simulink model "DualStreamSSR"  (R2023a)
settings: Solver=VariableStepAuto  StartTime=0.0  StopTime=4096  RelTol=1e-3
PreLoadFcn:
  | SSR4_init
InitFcn:
  | SSR4_init
undefined symbols (not defined in the file): DoubleStream, FIR_MultiKernel_cin, FIR_MultiKernel_cincout, FIR_MultiKernel_cout, N, S, SHIFT_ACC, Taps, vsva2197, xcvc1902
libraries: aieBasic x224, aieUtilities x16, dspsrcs4 x1, simulink x1, vmcUtilities x1
(part 2 of 6)

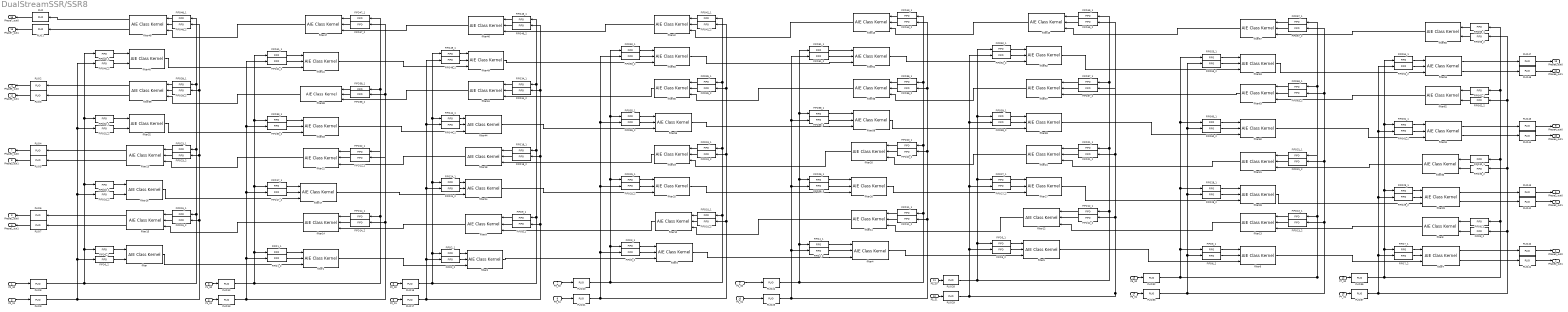
== system DualStreamSSR/SSR8 ==
  P0_S0 : Inport
  P0_S1 : Inport  Port=2
  P1_S0 : Inport  Port=3
  P1_S1 : Inport  Port=4
  P2_S0 : Inport  Port=5
  P2_S1 : Inport  Port=6
  P3_S0 : Inport  Port=7
  P3_S1 : Inport  Port=8
  P4_S0 : Inport  Port=9
  P4_S1 : Inport  Port=10
  P5_S0 : Inport  Port=11
  P5_S1 : Inport  Port=12
  P6_S0 : Inport  Port=13
  P6_S1 : Inport  Port=14
  P7_S0 : Inport  Port=15
  P7_S1 : Inport  Port=16
  FIFO0_1 : aieBasic/FIFO  FifoDepth=512  FIFOType=0  TileType=0  RowLocation=0  ColLocation=0  channel=0  blockJsonConstraints="[{\"type\":\"constraint\",\"constraintType\":\"location_fifo\",\"sid\":\"1153\",\"lhs\":{\"type\":\"location\",\"templParam\":\"fifo\",\"args\":{\"type\":\"fifo\",\"name\":\"DualStreamSSR/SSR8/FIFO0_1\",\"sid\":\"1153\"}},\"rhs\":{\"type\":\"fifogroup\",\"fifotype\":\"dma_fifo\",\"tiletype\":\"aie\",\"column\":{\"type\":\"evaluable\",\"expr\":\"23\",\"value\":23},\"row\":{\"type\":\"evaluable\",\"expr\":\"0\",\"value\":0},\"address\":{\"type\":\"evaluable\",\"expr\":\"0x0000\",\"value\":0},\"identifier\":\"0\",\"size\":{\"type\":\"evaluable\",\"expr\":\"512\",\"value\":512}},\"equality\":true}]"  deprecateConstraints=0
  FIFO0_2 : aieBasic/FIFO  FifoDepth=512  FIFOType=0  TileType=0  RowLocation=0  ColLocation=0  channel=0  blockJsonConstraints="[{\"type\":\"constraint\",\"constraintType\":\"location_fifo\",\"sid\":\"1154\",\"lhs\":{\"type\":\"location\",\"templParam\":\"fifo\",\"args\":{\"type\":\"fifo\",\"name\":\"DualStreamSSR/SSR8/FIFO0_2\",\"sid\":\"1154\"}},\"rhs\":{\"type\":\"fifogroup\",\"fifotype\":\"dma_fifo\",\"tiletype\":\"aie\",\"column\":{\"type\":\"evaluable\",\"expr\":\"23\",\"value\":23},\"row\":{\"type\":\"evaluable\",\"expr\":\"0\",\"value\":0},\"address\":{\"type\":\"evaluable\",\"expr\":\"0x2000\",\"value\":8192},\"identifier\":\"0\",\"size\":{\"type\":\"evaluable\",\"expr\":\"512\",\"value\":512}},\"equality\":true}]"  deprecateConstraints=0
  FIFO10_1 : aieBasic/FIFO  FifoDepth=512  FIFOType=0  TileType=0  RowLocation=0  ColLocation=0  channel=0  blockJsonConstraints="[{\"type\":\"constraint\",\"constraintType\":\"location_fifo\",\"sid\":\"1213\",\"lhs\":{\"type\":\"location\",\"templParam\":\"fifo\",\"args\":{\"type\":\"fifo\",\"name\":\"DualStreamSSR/SSR8/FIFO10_1\",\"sid\":\"1213\"}},\"rhs\":{\"type\":\"fifogroup\",\"fifotype\":\"dma_fifo\",\"tiletype\":\"aie\",\"column\":{\"type\":\"evaluable\",\"expr\":\"26\",\"value\":26},\"row\":{\"type\":\"evaluable\",\"expr\":\"1\",\"value\":1},\"address\":{\"type\":\"evaluable\",\"expr\":\"0x0000\",\"value\":0},\"identifier\":\"0\",\"size\":{\"type\":\"evaluable\",\"expr\":\"512\",\"value\":512}},\"equality\":true}]"  deprecateConstraints=0
  FIFO10_2 : aieBasic/FIFO  FifoDepth=512  FIFOType=0  TileType=0  RowLocation=0  ColLocation=0  channel=0  blockJsonConstraints="[{\"type\":\"constraint\",\"constraintType\":\"location_fifo\",\"sid\":\"1214\",\"lhs\":{\"type\":\"location\",\"templParam\":\"fifo\",\"args\":{\"type\":\"fifo\",\"name\":\"DualStreamSSR/SSR8/FIFO10_2\",\"sid\":\"1214\"}},\"rhs\":{\"type\":\"fifogroup\",\"fifotype\":\"dma_fifo\",\"tiletype\":\"aie\",\"column\":{\"type\":\"evaluable\",\"expr\":\"26\",\"value\":26},\"row\":{\"type\":\"evaluable\",\"expr\":\"1\",\"value\":1},\"address\":{\"type\":\"evaluable\",\"expr\":\"0x2000\",\"value\":8192},\"identifier\":\"0\",\"size\":{\"type\":\"evaluable\",\"expr\":\"512\",\"value\":512}},\"equality\":true}]"  deprecateConstraints=0
  FIFO11_1 : aieBasic/FIFO  FifoDepth=512  FIFOType=0  TileType=0  RowLocation=0  ColLocation=0  channel=0  blockJsonConstraints="[{\"type\":\"constraint\",\"constraintType\":\"location_fifo\",\"sid\":\"1229\",\"lhs\":{\"type\":\"location\",\"templParam\":\"fifo\",\"args\":{\"type\":\"fifo\",\"name\":\"DualStreamSSR/SSR8/FIFO11_1\",\"sid\":\"1229\"}},\"rhs\":{\"type\":\"fifogroup\",\"fifotype\":\"dma_fifo\",\"tiletype\":\"aie\",\"column\":{\"type\":\"evaluable\",\"expr\":\"27\",\"value\":27},\"row\":{\"type\":\"evaluable\",\"expr\":\"1\",\"value\":1},\"address\":{\"type\":\"evaluable\",\"expr\":\"0x0000\",\"value\":0},\"identifier\":\"0\",\"size\":{\"type\":\"evaluable\",\"expr\":\"512\",\"value\":512}},\"equality\":true}]"  deprecateConstraints=0
  FIFO11_2 : aieBasic/FIFO  FifoDepth=512  FIFOType=0  TileType=0  RowLocation=0  ColLocation=0  channel=0  blockJsonConstraints="[{\"type\":\"constraint\",\"constraintType\":\"location_fifo\",\"sid\":\"1230\",\"lhs\":{\"type\":\"location\",\"templParam\":\"fifo\",\"args\":{\"type\":\"fifo\",\"name\":\"DualStreamSSR/SSR8/FIFO11_2\",\"sid\":\"1230\"}},\"rhs\":{\"type\":\"fifogroup\",\"fifotype\":\"dma_fifo\",\"tiletype\":\"aie\",\"column\":{\"type\":\"evaluable\",\"expr\":\"27\",\"value\":27},\"row\":{\"type\":\"evaluable\",\"expr\":\"1\",\"value\":1},\"address\":{\"type\":\"evaluable\",\"expr\":\"0x2000\",\"value\":8192},\"identifier\":\"0\",\"size\":{\"type\":\"evaluable\",\"expr\":\"512\",\"value\":512}},\"equality\":true}]"  deprecateConstraints=0
  FIFO12_1 : aieBasic/FIFO  FifoDepth=512  FIFOType=0  TileType=0  RowLocation=0  ColLocation=0  channel=0  blockJsonConstraints="[{\"type\":\"constraint\",\"constraintType\":\"location_fifo\",\"sid\":\"1245\",\"lhs\":{\"type\":\"location\",\"templParam\":\"fifo\",\"args\":{\"type\":\"fifo\",\"name\":\"DualStreamSSR/SSR8/FIFO12_1\",\"sid\":\"1245\"}},\"rhs\":{\"type\":\"fifogroup\",\"fifotype\":\"dma_fifo\",\"tiletype\":\"aie\",\"column\":{\"type\":\"evaluable\",\"expr\":\"28\",\"value\":28},\"row\":{\"type\":\"evaluable\",\"expr\":\"1\",\"value\":1},\"address\":{\"type\":\"evaluable\",\"expr\":\"0x0000\",\"value\":0},\"identifier\":\"0\",\"size\":{\"type\":\"evaluable\",\"expr\":\"512\",\"value\":512}},\"equality\":true}]"  deprecateConstraints=0
  FIFO12_2 : aieBasic/FIFO  FifoDepth=512  FIFOType=0  TileType=0  RowLocation=0  ColLocation=0  channel=0  blockJsonConstraints="[{\"type\":\"constraint\",\"constraintType\":\"location_fifo\",\"sid\":\"1246\",\"lhs\":{\"type\":\"location\",\"templParam\":\"fifo\",\"args\":{\"type\":\"fifo\",\"name\":\"DualStreamSSR/SSR8/FIFO12_2\",\"sid\":\"1246\"}},\"rhs\":{\"type\":\"fifogroup\",\"fifotype\":\"dma_fifo\",\"tiletype\":\"aie\",\"column\":{\"type\":\"evaluable\",\"expr\":\"28\",\"value\":28},\"row\":{\"type\":\"evaluable\",\"expr\":\"1\",\"value\":1},\"address\":{\"type\":\"evaluable\",\"expr\":\"0x2000\",\"value\":8192},\"identifier\":\"0\",\"size\":{\"type\":\"evaluable\",\"expr\":\"512\",\"value\":512}},\"equality\":true}]"  deprecateConstraints=0
  FIFO13_1 : aieBasic/FIFO  FifoDepth=512  FIFOType=0  TileType=0  RowLocation=0  ColLocation=0  channel=0  blockJsonConstraints="[{\"type\":\"constraint\",\"constraintType\":\"location_fifo\",\"sid\":\"1261\",\"lhs\":{\"type\":\"location\",\"templParam\":\"fifo\",\"args\":{\"type\":\"fifo\",\"name\":\"DualStreamSSR/SSR8/FIFO13_1\",\"sid\":\"1261\"}},\"rhs\":{\"type\":\"fifogroup\",\"fifotype\":\"dma_fifo\",\"tiletype\":\"aie\",\"column\":{\"type\":\"evaluable\",\"expr\":\"29\",\"value\":29},\"row\":{\"type\":\"evaluable\",\"expr\":\"1\",\"value\":1},\"address\":{\"type\":\"evaluable\",\"expr\":\"0x0000\",\"value\":0},\"identifier\":\"0\",\"size\":{\"type\":\"evaluable\",\"expr\":\"512\",\"value\":512}},\"equality\":true}]"  deprecateConstraints=0
  FIFO13_2 : aieBasic/FIFO  FifoDepth=512  FIFOType=0  TileType=0  RowLocation=0  ColLocation=0  channel=0  blockJsonConstraints="[{\"type\":\"constraint\",\"constraintType\":\"location_fifo\",\"sid\":\"1262\",\"lhs\":{\"type\":\"location\",\"templParam\":\"fifo\",\"args\":{\"type\":\"fifo\",\"name\":\"DualStreamSSR/SSR8/FIFO13_2\",\"sid\":\"1262\"}},\"rhs\":{\"type\":\"fifogroup\",\"fifotype\":\"dma_fifo\",\"tiletype\":\"aie\",\"column\":{\"type\":\"evaluable\",\"expr\":\"29\",\"value\":29},\"row\":{\"type\":\"evaluable\",\"expr\":\"1\",\"value\":1},\"address\":{\"type\":\"evaluable\",\"expr\":\"0x2000\",\"value\":8192},\"identifier\":\"0\",\"size\":{\"type\":\"evaluable\",\"expr\":\"512\",\"value\":512}},\"equality\":true}]"  deprecateConstraints=0
  FIFO14_1 : aieBasic/FIFO  FifoDepth=512  FIFOType=0  TileType=0  RowLocation=0  ColLocation=0  channel=0  blockJsonConstraints="[{\"type\":\"constraint\",\"constraintType\":\"location_fifo\",\"sid\":\"1178\",\"lhs\":{\"type\":\"location\",\"templParam\":\"fifo\",\"args\":{\"type\":\"fifo\",\"name\":\"DualStreamSSR/SSR8/FIFO14_1\",\"sid\":\"1178\"}},\"rhs\":{\"type\":\"fifogroup\",\"fifotype\":\"dma_fifo\",\"tiletype\":\"aie\",\"column\":{\"type\":\"evaluable\",\"expr\":\"24\",\"value\":24},\"row\":{\"type\":\"evaluable\",\"expr\":\"1\",\"value\":1},\"address\":{\"type\":\"evaluable\",\"expr\":\"0x0000\",\"value\":0},\"identifier\":\"0\",\"size\":{\"type\":\"evaluable\",\"expr\":\"512\",\"value\":512}},\"equality\":true}]"  deprecateConstraints=0
  FIFO14_2 : aieBasic/FIFO  FifoDepth=512  FIFOType=0  TileType=0  RowLocation=0  ColLocation=0  channel=0  blockJsonConstraints="[{\"type\":\"constraint\",\"constraintType\":\"location_fifo\",\"sid\":\"1179\",\"lhs\":{\"type\":\"location\",\"templParam\":\"fifo\",\"args\":{\"type\":\"fifo\",\"name\":\"DualStreamSSR/SSR8/FIFO14_2\",\"sid\":\"1179\"}},\"rhs\":{\"type\":\"fifogroup\",\"fifotype\":\"dma_fifo\",\"tiletype\":\"aie\",\"column\":{\"type\":\"evaluable\",\"expr\":\"24\",\"value\":24},\"row\":{\"type\":\"evaluable\",\"expr\":\"1\",\"value\":1},\"address\":{\"type\":\"evaluable\",\"expr\":\"0x2000\",\"value\":8192},\"identifier\":\"0\",\"size\":{\"type\":\"evaluable\",\"expr\":\"512\",\"value\":512}},\"equality\":true}]"  deprecateConstraints=0
  FIFO15_1 : aieBasic/FIFO  FifoDepth=512  FIFOType=0  TileType=0  RowLocation=0  ColLocation=0  channel=0  blockJsonConstraints="[{\"type\":\"constraint\",\"constraintType\":\"location_fifo\",\"sid\":\"1162\",\"lhs\":{\"type\":\"location\",\"templParam\":\"fifo\",\"args\":{\"type\":\"fifo\",\"name\":\"DualStreamSSR/SSR8/FIFO15_1\",\"sid\":\"1162\"}},\"rhs\":{\"type\":\"fifogroup\",\"fifotype\":\"dma_fifo\",\"tiletype\":\"aie\",\"column\":{\"type\":\"evaluable\",\"expr\":\"23\",\"value\":23},\"row\":{\"type\":\"evaluable\",\"expr\":\"1\",\"value\":1},\"address\":{\"type\":\"evaluable\",\"expr\":\"0x0000\",\"value\":0},\"identifier\":\"0\",\"size\":{\"type\":\"evaluable\",\"expr\":\"512\",\"value\":512}},\"equality\":true}]"  deprecateConstraints=0
  FIFO15_2 : aieBasic/FIFO  FifoDepth=512  FIFOType=0  TileType=0  RowLocation=0  ColLocation=0  channel=0  blockJsonConstraints="[{\"type\":\"constraint\",\"constraintType\":\"location_fifo\",\"sid\":\"1163\",\"lhs\":{\"type\":\"location\",\"templParam\":\"fifo\",\"args\":{\"type\":\"fifo\",\"name\":\"DualStreamSSR/SSR8/FIFO15_2\",\"sid\":\"1163\"}},\"rhs\":{\"type\":\"fifogroup\",\"fifotype\":\"dma_fifo\",\"tiletype\":\"aie\",\"column\":{\"type\":\"evaluable\",\"expr\":\"23\",\"value\":23},\"row\":{\"type\":\"evaluable\",\"expr\":\"1\",\"value\":1},\"address\":{\"type\":\"evaluable\",\"expr\":\"0x2000\",\"value\":8192},\"identifier\":\"0\",\"size\":{\"type\":\"evaluable\",\"expr\":\"512\",\"value\":512}},\"equality\":true}]"  deprecateConstraints=0
  FIFO16_1 : aieBasic/FIFO  FifoDepth=512  FIFOType=0  TileType=0  RowLocation=0  ColLocation=0  channel=0  blockJsonConstraints="[{\"type\":\"constraint\",\"constraintType\":\"location_fifo\",\"sid\":\"1151\",\"lhs\":{\"type\":\"location\",\"templParam\":\"fifo\",\"args\":{\"type\":\"fifo\",\"name\":\"DualStreamSSR/SSR8/FIFO16_1\",\"sid\":\"1151\"}},\"rhs\":{\"type\":\"fifogroup\",\"fifotype\":\"dma_fifo\",\"tiletype\":\"aie\",\"column\":{\"type\":\"evaluable\",\"expr\":\"23\",\"value\":23},\"row\":{\"type\":\"evaluable\",\"expr\":\"2\",\"value\":2},\"address\":{\"type\":\"evaluable\",\"expr\":\"0x0000\",\"value\":0},\"identifier\":\"0\",\"size\":{\"type\":\"evaluable\",\"expr\":\"512\",\"value\":512}},\"equality\":true}]"  deprecateConstraints=0
  FIFO16_2 : aieBasic/FIFO  FifoDepth=512  FIFOType=0  TileType=0  RowLocation=0  ColLocation=0  channel=0  blockJsonConstraints="[{\"type\":\"constraint\",\"constraintType\":\"location_fifo\",\"sid\":\"1152\",\"lhs\":{\"type\":\"location\",\"templParam\":\"fifo\",\"args\":{\"type\":\"fifo\",\"name\":\"DualStreamSSR/SSR8/FIFO16_2\",\"sid\":\"1152\"}},\"rhs\":{\"type\":\"fifogroup\",\"fifotype\":\"dma_fifo\",\"tiletype\":\"aie\",\"column\":{\"type\":\"evaluable\",\"expr\":\"23\",\"value\":23},\"row\":{\"type\":\"evaluable\",\"expr\":\"2\",\"value\":2},\"address\":{\"type\":\"evaluable\",\"expr\":\"0x2000\",\"value\":8192},\"identifier\":\"0\",\"size\":{\"type\":\"evaluable\",\"expr\":\"512\",\"value\":512}},\"equality\":true}]"  deprecateConstraints=0
  FIFO17_1 : aieBasic/FIFO  FifoDepth=512  FIFOType=0  TileType=0  RowLocation=0  ColLocation=0  channel=0  blockJsonConstraints="[{\"type\":\"constraint\",\"constraintType\":\"location_fifo\",\"sid\":\"1168\",\"lhs\":{\"type\":\"location\",\"templParam\":\"fifo\",\"args\":{\"type\":\"fifo\",\"name\":\"DualStreamSSR/SSR8/FIFO17_1\",\"sid\":\"1168\"}},\"rhs\":{\"type\":\"fifogroup\",\"fifotype\":\"dma_fifo\",\"tiletype\":\"aie\",\"column\":{\"type\":\"evaluable\",\"expr\":\"24\",\"value\":24},\"row\":{\"type\":\"evaluable\",\"expr\":\"2\",\"value\":2},\"address\":{\"type\":\"evaluable\",\"expr\":\"0x0000\",\"value\":0},\"identifier\":\"0\",\"size\":{\"type\":\"evaluable\",\"expr\":\"512\",\"value\":512}},\"equality\":true}]"  deprecateConstraints=0
  FIFO17_2 : aieBasic/FIFO  FifoDepth=512  FIFOType=0  TileType=0  RowLocation=0  ColLocation=0  channel=0  blockJsonConstraints="[{\"type\":\"constraint\",\"constraintType\":\"location_fifo\",\"sid\":\"1169\",\"lhs\":{\"type\":\"location\",\"templParam\":\"fifo\",\"args\":{\"type\":\"fifo\",\"name\":\"DualStreamSSR/SSR8/FIFO17_2\",\"sid\":\"1169\"}},\"rhs\":{\"type\":\"fifogroup\",\"fifotype\":\"dma_fifo\",\"tiletype\":\"aie\",\"column\":{\"type\":\"evaluable\",\"expr\":\"24\",\"value\":24},\"row\":{\"type\":\"evaluable\",\"expr\":\"2\",\"value\":2},\"address\":{\"type\":\"evaluable\",\"expr\":\"0x2000\",\"value\":8192},\"identifier\":\"0\",\"size\":{\"type\":\"evaluable\",\"expr\":\"512\",\"value\":512}},\"equality\":true}]"  deprecateConstraints=0
  FIFO18_1 : aieBasic/FIFO  FifoDepth=512  FIFOType=0  TileType=0  RowLocation=0  ColLocation=0  channel=0  blockJsonConstraints="[{\"type\":\"constraint\",\"constraintType\":\"location_fifo\",\"sid\":\"1193\",\"lhs\":{\"type\":\"location\",\"templParam\":\"fifo\",\"args\":{\"type\":\"fifo\",\"name\":\"DualStreamSSR/SSR8/FIFO18_1\",\"sid\":\"1193\"}},\"rhs\":{\"type\":\"fifogroup\",\"fifotype\":\"dma_fifo\",\"tiletype\":\"aie\",\"column\":{\"type\":\"evaluable\",\"expr\":\"25\",\"value\":25},\"row\":{\"type\":\"evaluable\",\"expr\":\"3\",\"value\":3},\"address\":{\"type\":\"evaluable\",\"expr\":\"0x0000\",\"value\":0},\"identifier\":\"0\",\"size\":{\"type\":\"evaluable\",\"expr\":\"512\",\"value\":512}},\"equality\":true}]"  deprecateConstraints=0
  FIFO18_2 : aieBasic/FIFO  FifoDepth=512  FIFOType=0  TileType=0  RowLocation=0  ColLocation=0  channel=0  blockJsonConstraints="[{\"type\":\"constraint\",\"constraintType\":\"location_fifo\",\"sid\":\"1194\",\"lhs\":{\"type\":\"location\",\"templParam\":\"fifo\",\"args\":{\"type\":\"fifo\",\"name\":\"DualStreamSSR/SSR8/FIFO18_2\",\"sid\":\"1194\"}},\"rhs\":{\"type\":\"fifogroup\",\"fifotype\":\"dma_fifo\",\"tiletype\":\"aie\",\"column\":{\"type\":\"evaluable\",\"expr\":\"25\",\"value\":25},\"row\":{\"type\":\"evaluable\",\"expr\":\"3\",\"value\":3},\"address\":{\"type\":\"evaluable\",\"expr\":\"0x2000\",\"value\":8192},\"identifier\":\"0\",\"size\":{\"type\":\"evaluable\",\"expr\":\"512\",\"value\":512}},\"equality\":true}]"  deprecateConstraints=0
  FIFO19_1 : aieBasic/FIFO  FifoDepth=512  FIFOType=0  TileType=0  RowLocation=0  ColLocation=0  channel=0  blockJsonConstraints="[{\"type\":\"constraint\",\"constraintType\":\"location_fifo\",\"sid\":\"1211\",\"lhs\":{\"type\":\"location\",\"templParam\":\"fifo\",\"args\":{\"type\":\"fifo\",\"name\":\"DualStreamSSR/SSR8/FIFO19_1\",\"sid\":\"1211\"}},\"rhs\":{\"type\":\"fifogroup\",\"fifotype\":\"dma_fifo\",\"tiletype\":\"aie\",\"column\":{\"type\":\"evaluable\",\"expr\":\"26\",\"value\":26},\"row\":{\"type\":\"evaluable\",\"expr\":\"3\",\"value\":3},\"address\":{\"type\":\"evaluable\",\"expr\":\"0x0000\",\"value\":0},\"identifier\":\"0\",\"size\":{\"type\":\"evaluable\",\"expr\":\"512\",\"value\":512}},\"equality\":true}]"  deprecateConstraints=0
  FIFO19_2 : aieBasic/FIFO  FifoDepth=512  FIFOType=0  TileType=0  RowLocation=0  ColLocation=0  channel=0  blockJsonConstraints="[{\"type\":\"constraint\",\"constraintType\":\"location_fifo\",\"sid\":\"1212\",\"lhs\":{\"type\":\"location\",\"templParam\":\"fifo\",\"args\":{\"type\":\"fifo\",\"name\":\"DualStreamSSR/SSR8/FIFO19_2\",\"sid\":\"1212\"}},\"rhs\":{\"type\":\"fifogroup\",\"fifotype\":\"dma_fifo\",\"tiletype\":\"aie\",\"column\":{\"type\":\"evaluable\",\"expr\":\"26\",\"value\":26},\"row\":{\"type\":\"evaluable\",\"expr\":\"3\",\"value\":3},\"address\":{\"type\":\"evaluable\",\"expr\":\"0x2000\",\"value\":8192},\"identifier\":\"0\",\"size\":{\"type\":\"evaluable\",\"expr\":\"512\",\"value\":512}},\"equality\":true}]"  deprecateConstraints=0
  FIFO1_1 : aieBasic/FIFO  FifoDepth=512  FIFOType=0  TileType=0  RowLocation=0  ColLocation=0  channel=0  blockJsonConstraints="[{\"type\":\"constraint\",\"constraintType\":\"location_fifo\",\"sid\":\"1170\",\"lhs\":{\"type\":\"location\",\"templParam\":\"fifo\",\"args\":{\"type\":\"fifo\",\"name\":\"DualStreamSSR/SSR8/FIFO1_1\",\"sid\":\"1170\"}},\"rhs\":{\"type\":\"fifogroup\",\"fifotype\":\"dma_fifo\",\"tiletype\":\"aie\",\"column\":{\"type\":\"evaluable\",\"expr\":\"24\",\"value\":24},\"row\":{\"type\":\"evaluable\",\"expr\":\"0\",\"value\":0},\"address\":{\"type\":\"evaluable\",\"expr\":\"0x0000\",\"value\":0},\"identifier\":\"0\",\"size\":{\"type\":\"evaluable\",\"expr\":\"512\",\"value\":512}},\"equality\":true}]"  deprecateConstraints=0
  FIFO1_2 : aieBasic/FIFO  FifoDepth=512  FIFOType=0  TileType=0  RowLocation=0  ColLocation=0  channel=0  blockJsonConstraints="[{\"type\":\"constraint\",\"constraintType\":\"location_fifo\",\"sid\":\"1171\",\"lhs\":{\"type\":\"location\",\"templParam\":\"fifo\",\"args\":{\"type\":\"fifo\",\"name\":\"DualStreamSSR/SSR8/FIFO1_2\",\"sid\":\"1171\"}},\"rhs\":{\"type\":\"fifogroup\",\"fifotype\":\"dma_fifo\",\"tiletype\":\"aie\",\"column\":{\"type\":\"evaluable\",\"expr\":\"24\",\"value\":24},\"row\":{\"type\":\"evaluable\",\"expr\":\"0\",\"value\":0},\"address\":{\"type\":\"evaluable\",\"expr\":\"0x2000\",\"value\":8192},\"identifier\":\"0\",\"size\":{\"type\":\"evaluable\",\"expr\":\"512\",\"value\":512}},\"equality\":true}]"  deprecateConstraints=0
  FIFO20_1 : aieBasic/FIFO  FifoDepth=512  FIFOType=0  TileType=0  RowLocation=0  ColLocation=0  channel=0  blockJsonConstraints="[{\"type\":\"constraint\",\"constraintType\":\"location_fifo\",\"sid\":\"1227\",\"lhs\":{\"type\":\"location\",\"templParam\":\"fifo\",\"args\":{\"type\":\"fifo\",\"name\":\"DualStreamSSR/SSR8/FIFO20_1\",\"sid\":\"1227\"}},\"rhs\":{\"type\":\"fifogroup\",\"fifotype\":\"dma_fifo\",\"tiletype\":\"aie\",\"column\":{\"type\":\"evaluable\",\"expr\":\"27\",\"value\":27},\"row\":{\"type\":\"evaluable\",\"expr\":\"3\",\"value\":3},\"address\":{\"type\":\"evaluable\",\"expr\":\"0x0000\",\"value\":0},\"identifier\":\"0\",\"size\":{\"type\":\"evaluable\",\"expr\":\"512\",\"value\":512}},\"equality\":true}]"  deprecateConstraints=0
  FIFO20_2 : aieBasic/FIFO  FifoDepth=512  FIFOType=0  TileType=0  RowLocation=0  ColLocation=0  channel=0  blockJsonConstraints="[{\"type\":\"constraint\",\"constraintType\":\"location_fifo\",\"sid\":\"1228\",\"lhs\":{\"type\":\"location\",\"templParam\":\"fifo\",\"args\":{\"type\":\"fifo\",\"name\":\"DualStreamSSR/SSR8/FIFO20_2\",\"sid\":\"1228\"}},\"rhs\":{\"type\":\"fifogroup\",\"fifotype\":\"dma_fifo\",\"tiletype\":\"aie\",\"column\":{\"type\":\"evaluable\",\"expr\":\"27\",\"value\":27},\"row\":{\"type\":\"evaluable\",\"expr\":\"3\",\"value\":3},\"address\":{\"type\":\"evaluable\",\"expr\":\"0x2000\",\"value\":8192},\"identifier\":\"0\",\"size\":{\"type\":\"evaluable\",\"expr\":\"512\",\"value\":512}},\"equality\":true}]"  deprecateConstraints=0
  FIFO21_1 : aieBasic/FIFO  FifoDepth=512  FIFOType=0  TileType=0  RowLocation=0  ColLocation=0  channel=0  blockJsonConstraints="[{\"type\":\"constraint\",\"constraintType\":\"location_fifo\",\"sid\":\"1243\",\"lhs\":{\"type\":\"location\",\"templParam\":\"fifo\",\"args\":{\"type\":\"fifo\",\"name\":\"DualStreamSSR/SSR8/FIFO21_1\",\"sid\":\"1243\"}},\"rhs\":{\"type\":\"fifogroup\",\"fifotype\":\"dma_fifo\",\"tiletype\":\"aie\",\"column\":{\"type\":\"evaluable\",\"expr\":\"28\",\"value\":28},\"row\":{\"type\":\"evaluable\",\"expr\":\"3\",\"value\":3},\"address\":{\"type\":\"evaluable\",\"expr\":\"0x0000\",\"value\":0},\"identifier\":\"0\",\"size\":{\"type\":\"evaluable\",\"expr\":\"512\",\"value\":512}},\"equality\":true}]"  deprecateConstraints=0
  FIFO21_2 : aieBasic/FIFO  FifoDepth=512  FIFOType=0  TileType=0  RowLocation=0  ColLocation=0  channel=0  blockJsonConstraints="[{\"type\":\"constraint\",\"constraintType\":\"location_fifo\",\"sid\":\"1244\",\"lhs\":{\"type\":\"location\",\"templParam\":\"fifo\",\"args\":{\"type\":\"fifo\",\"name\":\"DualStreamSSR/SSR8/FIFO21_2\",\"sid\":\"1244\"}},\"rhs\":{\"type\":\"fifogroup\",\"fifotype\":\"dma_fifo\",\"tiletype\":\"aie\",\"column\":{\"type\":\"evaluable\",\"expr\":\"28\",\"value\":28},\"row\":{\"type\":\"evaluable\",\"expr\":\"3\",\"value\":3},\"address\":{\"type\":\"evaluable\",\"expr\":\"0x2000\",\"value\":8192},\"identifier\":\"0\",\"size\":{\"type\":\"evaluable\",\"expr\":\"512\",\"value\":512}},\"equality\":true}]"  deprecateConstraints=0
  FIFO22_1 : aieBasic/FIFO  FifoDepth=512  FIFOType=0  TileType=0  RowLocation=0  ColLocation=0  channel=0  blockJsonConstraints="[{\"type\":\"constraint\",\"constraintType\":\"location_fifo\",\"sid\":\"1176\",\"lhs\":{\"type\":\"location\",\"templParam\":\"fifo\",\"args\":{\"type\":\"fifo\",\"name\":\"DualStreamSSR/SSR8/FIFO22_1\",\"sid\":\"1176\"}},\"rhs\":{\"type\":\"fifogroup\",\"fifotype\":\"dma_fifo\",\"tiletype\":\"aie\",\"column\":{\"type\":\"evaluable\",\"expr\":\"24\",\"value\":24},\"row\":{\"type\":\"evaluable\",\"expr\":\"3\",\"value\":3},\"address\":{\"type\":\"evaluable\",\"expr\":\"0x0000\",\"value\":0},\"identifier\":\"0\",\"size\":{\"type\":\"evaluable\",\"expr\":\"512\",\"value\":512}},\"equality\":true}]"  deprecateConstraints=0
  FIFO22_2 : aieBasic/FIFO  FifoDepth=512  FIFOType=0  TileType=0  RowLocation=0  ColLocation=0  channel=0  blockJsonConstraints="[{\"type\":\"constraint\",\"constraintType\":\"location_fifo\",\"sid\":\"1177\",\"lhs\":{\"type\":\"location\",\"templParam\":\"fifo\",\"args\":{\"type\":\"fifo\",\"name\":\"DualStreamSSR/SSR8/FIFO22_2\",\"sid\":\"1177\"}},\"rhs\":{\"type\":\"fifogroup\",\"fifotype\":\"dma_fifo\",\"tiletype\":\"aie\",\"column\":{\"type\":\"evaluable\",\"expr\":\"24\",\"value\":24},\"row\":{\"type\":\"evaluable\",\"expr\":\"3\",\"value\":3},\"address\":{\"type\":\"evaluable\",\"expr\":\"0x2000\",\"value\":8192},\"identifier\":\"0\",\"size\":{\"type\":\"evaluable\",\"expr\":\"512\",\"value\":512}},\"equality\":true}]"  deprecateConstraints=0
  FIFO23_1 : aieBasic/FIFO  FifoDepth=512  FIFOType=0  TileType=0  RowLocation=0  ColLocation=0  channel=0  blockJsonConstraints="[{\"type\":\"constraint\",\"constraintType\":\"location_fifo\",\"sid\":\"1160\",\"lhs\":{\"type\":\"location\",\"templParam\":\"fifo\",\"args\":{\"type\":\"fifo\",\"name\":\"DualStreamSSR/SSR8/FIFO23_1\",\"sid\":\"1160\"}},\"rhs\":{\"type\":\"fifogroup\",\"fifotype\":\"dma_fifo\",\"tiletype\":\"aie\",\"column\":{\"type\":\"evaluable\",\"expr\":\"23\",\"value\":23},\"row\":{\"type\":\"evaluable\",\"expr\":\"3\",\"value\":3},\"address\":{\"type\":\"evaluable\",\"expr\":\"0x0000\",\"value\":0},\"identifier\":\"0\",\"size\":{\"type\":\"evaluable\",\"expr\":\"512\",\"value\":512}},\"equality\":true}]"  deprecateConstraints=0
  FIFO23_2 : aieBasic/FIFO  FifoDepth=512  FIFOType=0  TileType=0  RowLocation=0  ColLocation=0  channel=0  blockJsonConstraints="[{\"type\":\"constraint\",\"constraintType\":\"location_fifo\",\"sid\":\"1161\",\"lhs\":{\"type\":\"location\",\"templParam\":\"fifo\",\"args\":{\"type\":\"fifo\",\"name\":\"DualStreamSSR/SSR8/FIFO23_2\",\"sid\":\"1161\"}},\"rhs\":{\"type\":\"fifogroup\",\"fifotype\":\"dma_fifo\",\"tiletype\":\"aie\",\"column\":{\"type\":\"evaluable\",\"expr\":\"23\",\"value\":23},\"row\":{\"type\":\"evaluable\",\"expr\":\"3\",\"value\":3},\"address\":{\"type\":\"evaluable\",\"expr\":\"0x2000\",\"value\":8192},\"identifier\":\"0\",\"size\":{\"type\":\"evaluable\",\"expr\":\"512\",\"value\":512}},\"equality\":true}]"  deprecateConstraints=0
  FIFO24_1 : aieBasic/FIFO  FifoDepth=512  FIFOType=0  TileType=0  RowLocation=0  ColLocation=0  channel=0  blockJsonConstraints="[{\"type\":\"constraint\",\"constraintType\":\"location_fifo\",\"sid\":\"1184\",\"lhs\":{\"type\":\"location\",\"templParam\":\"fifo\",\"args\":{\"type\":\"fifo\",\"name\":\"DualStreamSSR/SSR8/FIFO24_1\",\"sid\":\"1184\"}},\"rhs\":{\"type\":\"fifogroup\",\"fifotype\":\"dma_fifo\",\"tiletype\":\"aie\",\"column\":{\"type\":\"evaluable\",\"expr\":\"25\",\"value\":25},\"row\":{\"type\":\"evaluable\",\"expr\":\"2\",\"value\":2},\"address\":{\"type\":\"evaluable\",\"expr\":\"0x0000\",\"value\":0},\"identifier\":\"0\",\"size\":{\"type\":\"evaluable\",\"expr\":\"512\",\"value\":512}},\"equality\":true}]"  deprecateConstraints=0
  FIFO24_2 : aieBasic/FIFO  FifoDepth=512  FIFOType=0  TileType=0  RowLocation=0  ColLocation=0  channel=0  blockJsonConstraints="[{\"type\":\"constraint\",\"constraintType\":\"location_fifo\",\"sid\":\"1185\",\"lhs\":{\"type\":\"location\",\"templParam\":\"fifo\",\"args\":{\"type\":\"fifo\",\"name\":\"DualStreamSSR/SSR8/FIFO24_2\",\"sid\":\"1185\"}},\"rhs\":{\"type\":\"fifogroup\",\"fifotype\":\"dma_fifo\",\"tiletype\":\"aie\",\"column\":{\"type\":\"evaluable\",\"expr\":\"25\",\"value\":25},\"row\":{\"type\":\"evaluable\",\"expr\":\"2\",\"value\":2},\"address\":{\"type\":\"evaluable\",\"expr\":\"0x2000\",\"value\":8192},\"identifier\":\"0\",\"size\":{\"type\":\"evaluable\",\"expr\":\"512\",\"value\":512}},\"equality\":true}]"  deprecateConstraints=0
  FIFO25_1 : aieBasic/FIFO  FifoDepth=512  FIFOType=0  TileType=0  RowLocation=0  ColLocation=0  channel=0  blockJsonConstraints="[{\"type\":\"constraint\",\"constraintType\":\"location_fifo\",\"sid\":\"1203\",\"lhs\":{\"type\":\"location\",\"templParam\":\"fifo\",\"args\":{\"type\":\"fifo\",\"name\":\"DualStreamSSR/SSR8/FIFO25_1\",\"sid\":\"1203\"}},\"rhs\":{\"type\":\"fifogroup\",\"fifotype\":\"dma_fifo\",\"tiletype\":\"aie\",\"column\":{\"type\":\"evaluable\",\"expr\":\"26\",\"value\":26},\"row\":{\"type\":\"evaluable\",\"expr\":\"2\",\"value\":2},\"address\":{\"type\":\"evaluable\",\"expr\":\"0x0000\",\"value\":0},\"identifier\":\"0\",\"size\":{\"type\":\"evaluable\",\"expr\":\"512\",\"value\":512}},\"equality\":true}]"  deprecateConstraints=0
  FIFO25_2 : aieBasic/FIFO  FifoDepth=512  FIFOType=0  TileType=0  RowLocation=0  ColLocation=0  channel=0  blockJsonConstraints="[{\"type\":\"constraint\",\"constraintType\":\"location_fifo\",\"sid\":\"1204\",\"lhs\":{\"type\":\"location\",\"templParam\":\"fifo\",\"args\":{\"type\":\"fifo\",\"name\":\"DualStreamSSR/SSR8/FIFO25_2\",\"sid\":\"1204\"}},\"rhs\":{\"type\":\"fifogroup\",\"fifotype\":\"dma_fifo\",\"tiletype\":\"aie\",\"column\":{\"type\":\"evaluable\",\"expr\":\"26\",\"value\":26},\"row\":{\"type\":\"evaluable\",\"expr\":\"2\",\"value\":2},\"address\":{\"type\":\"evaluable\",\"expr\":\"0x2000\",\"value\":8192},\"identifier\":\"0\",\"size\":{\"type\":\"evaluable\",\"expr\":\"512\",\"value\":512}},\"equality\":true}]"  deprecateConstraints=0
  FIFO26_1 : aieBasic/FIFO  FifoDepth=512  FIFOType=0  TileType=0  RowLocation=0  ColLocation=0  channel=0  blockJsonConstraints="[{\"type\":\"constraint\",\"constraintType\":\"location_fifo\",\"sid\":\"1219\",\"lhs\":{\"type\":\"location\",\"templParam\":\"fifo\",\"args\":{\"type\":\"fifo\",\"name\":\"DualStreamSSR/SSR8/FIFO26_1\",\"sid\":\"1219\"}},\"rhs\":{\"type\":\"fifogroup\",\"fifotype\":\"dma_fifo\",\"tiletype\":\"aie\",\"column\":{\"type\":\"evaluable\",\"expr\":\"27\",\"value\":27},\"row\":{\"type\":\"evaluable\",\"expr\":\"2\",\"value\":2},\"address\":{\"type\":\"evaluable\",\"expr\":\"0x0000\",\"value\":0},\"identifier\":\"0\",\"size\":{\"type\":\"evaluable\",\"expr\":\"512\",\"value\":512}},\"equality\":true}]"  deprecateConstraints=0
  FIFO26_2 : aieBasic/FIFO  FifoDepth=512  FIFOType=0  TileType=0  RowLocation=0  ColLocation=0  channel=0  blockJsonConstraints="[{\"type\":\"constraint\",\"constraintType\":\"location_fifo\",\"sid\":\"1220\",\"lhs\":{\"type\":\"location\",\"templParam\":\"fifo\",\"args\":{\"type\":\"fifo\",\"name\":\"DualStreamSSR/SSR8/FIFO26_2\",\"sid\":\"1220\"}},\"rhs\":{\"type\":\"fifogroup\",\"fifotype\":\"dma_fifo\",\"tiletype\":\"aie\",\"column\":{\"type\":\"evaluable\",\"expr\":\"27\",\"value\":27},\"row\":{\"type\":\"evaluable\",\"expr\":\"2\",\"value\":2},\"address\":{\"type\":\"evaluable\",\"expr\":\"0x2000\",\"value\":8192},\"identifier\":\"0\",\"size\":{\"type\":\"evaluable\",\"expr\":\"512\",\"value\":512}},\"equality\":true}]"  deprecateConstraints=0
  FIFO27_1 : aieBasic/FIFO  FifoDepth=512  FIFOType=0  TileType=0  RowLocation=0  ColLocation=0  channel=0  blockJsonConstraints="[{\"type\":\"constraint\",\"constraintType\":\"location_fifo\",\"sid\":\"1235\",\"lhs\":{\"type\":\"location\",\"templParam\":\"fifo\",\"args\":{\"type\":\"fifo\",\"name\":\"DualStreamSSR/SSR8/FIFO27_1\",\"sid\":\"1235\"}},\"rhs\":{\"type\":\"fifogroup\",\"fifotype\":\"dma_fifo\",\"tiletype\":\"aie\",\"column\":{\"type\":\"evaluable\",\"expr\":\"28\",\"value\":28},\"row\":{\"type\":\"evaluable\",\"expr\":\"2\",\"value\":2},\"address\":{\"type\":\"evaluable\",\"expr\":\"0x0000\",\"value\":0},\"identifier\":\"0\",\"size\":{\"type\":\"evaluable\",\"expr\":\"512\",\"value\":512}},\"equality\":true}]"  deprecateConstraints=0
  FIFO27_2 : aieBasic/FIFO  FifoDepth=512  FIFOType=0  TileType=0  RowLocation=0  ColLocation=0  channel=0  blockJsonConstraints="[{\"type\":\"constraint\",\"constraintType\":\"location_fifo\",\"sid\":\"1236\",\"lhs\":{\"type\":\"location\",\"templParam\":\"fifo\",\"args\":{\"type\":\"fifo\",\"name\":\"DualStreamSSR/SSR8/FIFO27_2\",\"sid\":\"1236\"}},\"rhs\":{\"type\":\"fifogroup\",\"fifotype\":\"dma_fifo\",\"tiletype\":\"aie\",\"column\":{\"type\":\"evaluable\",\"expr\":\"28\",\"value\":28},\"row\":{\"type\":\"evaluable\",\"expr\":\"2\",\"value\":2},\"address\":{\"type\":\"evaluable\",\"expr\":\"0x2000\",\"value\":8192},\"identifier\":\"0\",\"size\":{\"type\":\"evaluable\",\"expr\":\"512\",\"value\":512}},\"equality\":true}]"  deprecateConstraints=0
  FIFO28_1 : aieBasic/FIFO  FifoDepth=512  FIFOType=0  TileType=0  RowLocation=0  ColLocation=0  channel=0  blockJsonConstraints="[{\"type\":\"constraint\",\"constraintType\":\"location_fifo\",\"sid\":\"1251\",\"lhs\":{\"type\":\"location\",\"templParam\":\"fifo\",\"args\":{\"type\":\"fifo\",\"name\":\"DualStreamSSR/SSR8/FIFO28_1\",\"sid\":\"1251\"}},\"rhs\":{\"type\":\"fifogroup\",\"fifotype\":\"dma_fifo\",\"tiletype\":\"aie\",\"column\":{\"type\":\"evaluable\",\"expr\":\"29\",\"value\":29},\"row\":{\"type\":\"evaluable\",\"expr\":\"2\",\"value\":2},\"address\":{\"type\":\"evaluable\",\"expr\":\"0x0000\",\"value\":0},\"identifier\":\"0\",\"size\":{\"type\":\"evaluable\",\"expr\":\"512\",\"value\":512}},\"equality\":true}]"  deprecateConstraints=0
  FIFO28_2 : aieBasic/FIFO  FifoDepth=512  FIFOType=0  TileType=0  RowLocation=0  ColLocation=0  channel=0  blockJsonConstraints="[{\"type\":\"constraint\",\"constraintType\":\"location_fifo\",\"sid\":\"1252\",\"lhs\":{\"type\":\"location\",\"templParam\":\"fifo\",\"args\":{\"type\":\"fifo\",\"name\":\"DualStreamSSR/SSR8/FIFO28_2\",\"sid\":\"1252\"}},\"rhs\":{\"type\":\"fifogroup\",\"fifotype\":\"dma_fifo\",\"tiletype\":\"aie\",\"column\":{\"type\":\"evaluable\",\"expr\":\"29\",\"value\":29},\"row\":{\"type\":\"evaluable\",\"expr\":\"2\",\"value\":2},\"address\":{\"type\":\"evaluable\",\"expr\":\"0x2000\",\"value\":8192},\"identifier\":\"0\",\"size\":{\"type\":\"evaluable\",\"expr\":\"512\",\"value\":512}},\"equality\":true}]"  deprecateConstraints=0
  FIFO29_1 : aieBasic/FIFO  FifoDepth=512  FIFOType=0  TileType=0  RowLocation=0  ColLocation=0  channel=0  blockJsonConstraints="[{\"type\":\"constraint\",\"constraintType\":\"location_fifo\",\"sid\":\"1267\",\"lhs\":{\"type\":\"location\",\"templParam\":\"fifo\",\"args\":{\"type\":\"fifo\",\"name\":\"DualStreamSSR/SSR8/FIFO29_1\",\"sid\":\"1267\"}},\"rhs\":{\"type\":\"fifogroup\",\"fifotype\":\"dma_fifo\",\"tiletype\":\"aie\",\"column\":{\"type\":\"evaluable\",\"expr\":\"30\",\"value\":30},\"row\":{\"type\":\"evaluable\",\"expr\":\"2\",\"value\":2},\"address\":{\"type\":\"evaluable\",\"expr\":\"0x0000\",\"value\":0},\"identifier\":\"0\",\"size\":{\"type\":\"evaluable\",\"expr\":\"512\",\"value\":512}},\"equality\":true}]"  deprecateConstraints=0
  FIFO29_2 : aieBasic/FIFO  FifoDepth=512  FIFOType=0  TileType=0  RowLocation=0  ColLocation=0  channel=0  blockJsonConstraints="[{\"type\":\"constraint\",\"constraintType\":\"location_fifo\",\"sid\":\"1268\",\"lhs\":{\"type\":\"location\",\"templParam\":\"fifo\",\"args\":{\"type\":\"fifo\",\"name\":\"DualStreamSSR/SSR8/FIFO29_2\",\"sid\":\"1268\"}},\"rhs\":{\"type\":\"fifogroup\",\"fifotype\":\"dma_fifo\",\"tiletype\":\"aie\",\"column\":{\"type\":\"evaluable\",\"expr\":\"30\",\"value\":30},\"row\":{\"type\":\"evaluable\",\"expr\":\"2\",\"value\":2},\"address\":{\"type\":\"evaluable\",\"expr\":\"0x2000\",\"value\":8192},\"identifier\":\"0\",\"size\":{\"type\":\"evaluable\",\"expr\":\"512\",\"value\":512}},\"equality\":true}]"  deprecateConstraints=0
  FIFO2_1 : aieBasic/FIFO  FifoDepth=512  FIFOType=0  TileType=0  RowLocation=0  ColLocation=0  channel=0  blockJsonConstraints="[{\"type\":\"constraint\",\"constraintType\":\"location_fifo\",\"sid\":\"1186\",\"lhs\":{\"type\":\"location\",\"templParam\":\"fifo\",\"args\":{\"type\":\"fifo\",\"name\":\"DualStreamSSR/SSR8/FIFO2_1\",\"sid\":\"1186\"}},\"rhs\":{\"type\":\"fifogroup\",\"fifotype\":\"dma_fifo\",\"tiletype\":\"aie\",\"column\":{\"type\":\"evaluable\",\"expr\":\"25\",\"value\":25},\"row\":{\"type\":\"evaluable\",\"expr\":\"0\",\"value\":0},\"address\":{\"type\":\"evaluable\",\"expr\":\"0x0000\",\"value\":0},\"identifier\":\"0\",\"size\":{\"type\":\"evaluable\",\"expr\":\"512\",\"value\":512}},\"equality\":true}]"  deprecateConstraints=0
  FIFO2_2 : aieBasic/FIFO  FifoDepth=512  FIFOType=0  TileType=0  RowLocation=0  ColLocation=0  channel=0  blockJsonConstraints="[{\"type\":\"constraint\",\"constraintType\":\"location_fifo\",\"sid\":\"1187\",\"lhs\":{\"type\":\"location\",\"templParam\":\"fifo\",\"args\":{\"type\":\"fifo\",\"name\":\"DualStreamSSR/SSR8/FIFO2_2\",\"sid\":\"1187\"}},\"rhs\":{\"type\":\"fifogroup\",\"fifotype\":\"dma_fifo\",\"tiletype\":\"aie\",\"column\":{\"type\":\"evaluable\",\"expr\":\"25\",\"value\":25},\"row\":{\"type\":\"evaluable\",\"expr\":\"0\",\"value\":0},\"address\":{\"type\":\"evaluable\",\"expr\":\"0x2000\",\"value\":8192},\"identifier\":\"0\",\"size\":{\"type\":\"evaluable\",\"expr\":\"512\",\"value\":512}},\"equality\":true}]"  deprecateConstraints=0
  FIFO30_1 : aieBasic/FIFO  FifoDepth=512  FIFOType=0  TileType=0  RowLocation=0  ColLocation=0  channel=0  blockJsonConstraints="[{\"type\":\"constraint\",\"constraintType\":\"location_fifo\",\"sid\":\"1275\",\"lhs\":{\"type\":\"location\",\"templParam\":\"fifo\",\"args\":{\"type\":\"fifo\",\"name\":\"DualStreamSSR/SSR8/FIFO30_1\",\"sid\":\"1275\"}},\"rhs\":{\"type\":\"fifogroup\",\"fifotype\":\"dma_fifo\",\"tiletype\":\"aie\",\"column\":{\"type\":\"evaluable\",\"expr\":\"30\",\"value\":30},\"row\":{\"type\":\"evaluable\",\"expr\":\"3\",\"value\":3},\"address\":{\"type\":\"evaluable\",\"expr\":\"0x0000\",\"value\":0},\"identifier\":\"0\",\"size\":{\"type\":\"evaluable\",\"expr\":\"512\",\"value\":512}},\"equality\":true}]"  deprecateConstraints=0
  FIFO30_2 : aieBasic/FIFO  FifoDepth=512  FIFOType=0  TileType=0  RowLocation=0  ColLocation=0  channel=0  blockJsonConstraints="[{\"type\":\"constraint\",\"constraintType\":\"location_fifo\",\"sid\":\"1276\",\"lhs\":{\"type\":\"location\",\"templParam\":\"fifo\",\"args\":{\"type\":\"fifo\",\"name\":\"DualStreamSSR/SSR8/FIFO30_2\",\"sid\":\"1276\"}},\"rhs\":{\"type\":\"fifogroup\",\"fifotype\":\"dma_fifo\",\"tiletype\":\"aie\",\"column\":{\"type\":\"evaluable\",\"expr\":\"30\",\"value\":30},\"row\":{\"type\":\"evaluable\",\"expr\":\"3\",\"value\":3},\"address\":{\"type\":\"evaluable\",\"expr\":\"0x2000\",\"value\":8192},\"identifier\":\"0\",\"size\":{\"type\":\"evaluable\",\"expr\":\"512\",\"value\":512}},\"equality\":true}]"  deprecateConstraints=0
  FIFO31_1 : aieBasic/FIFO  FifoDepth=512  FIFOType=0  TileType=0  RowLocation=0  ColLocation=0  channel=0  blockJsonConstraints="[{\"type\":\"constraint\",\"constraintType\":\"location_fifo\",\"sid\":\"1259\",\"lhs\":{\"type\":\"location\",\"templParam\":\"fifo\",\"args\":{\"type\":\"fifo\",\"name\":\"DualStreamSSR/SSR8/FIFO31_1\",\"sid\":\"1259\"}},\"rhs\":{\"type\":\"fifogroup\",\"fifotype\":\"dma_fifo\",\"tiletype\":\"aie\",\"column\":{\"type\":\"evaluable\",\"expr\":\"29\",\"value\":29},\"row\":{\"type\":\"evaluable\",\"expr\":\"3\",\"value\":3},\"address\":{\"type\":\"evaluable\",\"expr\":\"0x0000\",\"value\":0},\"identifier\":\"0\",\"size\":{\"type\":\"evaluable\",\"expr\":\"512\",\"value\":512}},\"equality\":true}]"  deprecateConstraints=0
  FIFO31_2 : aieBasic/FIFO  FifoDepth=512  FIFOType=0  TileType=0  RowLocation=0  ColLocation=0  channel=0  blockJsonConstraints="[{\"type\":\"constraint\",\"constraintType\":\"location_fifo\",\"sid\":\"1260\",\"lhs\":{\"type\":\"location\",\"templParam\":\"fifo\",\"args\":{\"type\":\"fifo\",\"name\":\"DualStreamSSR/SSR8/FIFO31_2\",\"sid\":\"1260\"}},\"rhs\":{\"type\":\"fifogroup\",\"fifotype\":\"dma_fifo\",\"tiletype\":\"aie\",\"column\":{\"type\":\"evaluable\",\"expr\":\"29\",\"value\":29},\"row\":{\"type\":\"evaluable\",\"expr\":\"3\",\"value\":3},\"address\":{\"type\":\"evaluable\",\"expr\":\"0x2000\",\"value\":8192},\"identifier\":\"0\",\"size\":{\"type\":\"evaluable\",\"expr\":\"512\",\"value\":512}},\"equality\":true}]"  deprecateConstraints=0
  FIFO32_1 : aieBasic/FIFO  FifoDepth=512  FIFOType=0  TileType=0  RowLocation=0  ColLocation=0  channel=0  blockJsonConstraints="[{\"type\":\"constraint\",\"constraintType\":\"location_fifo\",\"sid\":\"1149\",\"lhs\":{\"type\":\"location\",\"templParam\":\"fifo\",\"args\":{\"type\":\"fifo\",\"name\":\"DualStreamSSR/SSR8/FIFO32_1\",\"sid\":\"1149\"}},\"rhs\":{\"type\":\"fifogroup\",\"fifotype\":\"dma_fifo\",\"tiletype\":\"aie\",\"column\":{\"type\":\"evaluable\",\"expr\":\"23\",\"value\":23},\"row\":{\"type\":\"evaluable\",\"expr\":\"4\",\"value\":4},\"address\":{\"type\":\"evaluable\",\"expr\":\"0x0000\",\"value\":0},\"identifier\":\"0\",\"size\":{\"type\":\"evaluable\",\"expr\":\"512\",\"value\":512}},\"equality\":true}]"  deprecateConstraints=0
  FIFO32_2 : aieBasic/FIFO  FifoDepth=512  FIFOType=0  TileType=0  RowLocation=0  ColLocation=0  channel=0  blockJsonConstraints="[{\"type\":\"constraint\",\"constraintType\":\"location_fifo\",\"sid\":\"1150\",\"lhs\":{\"type\":\"location\",\"templParam\":\"fifo\",\"args\":{\"type\":\"fifo\",\"name\":\"DualStreamSSR/SSR8/FIFO32_2\",\"sid\":\"1150\"}},\"rhs\":{\"type\":\"fifogroup\",\"fifotype\":\"dma_fifo\",\"tiletype\":\"aie\",\"column\":{\"type\":\"evaluable\",\"expr\":\"23\",\"value\":23},\"row\":{\"type\":\"evaluable\",\"expr\":\"4\",\"value\":4},\"address\":{\"type\":\"evaluable\",\"expr\":\"0x2000\",\"value\":8192},\"identifier\":\"0\",\"size\":{\"type\":\"evaluable\",\"expr\":\"512\",\"value\":512}},\"equality\":true}]"  deprecateConstraints=0
  FIFO33_1 : aieBasic/FIFO  FifoDepth=512  FIFOType=0  TileType=0  RowLocation=0  ColLocation=0  channel=0  blockJsonConstraints="[{\"type\":\"constraint\",\"constraintType\":\"location_fifo\",\"sid\":\"1166\",\"lhs\":{\"type\":\"location\",\"templParam\":\"fifo\",\"args\":{\"type\":\"fifo\",\"name\":\"DualStreamSSR/SSR8/FIFO33_1\",\"sid\":\"1166\"}},\"rhs\":{\"type\":\"fifogroup\",\"fifotype\":\"dma_fifo\",\"tiletype\":\"aie\",\"column\":{\"type\":\"evaluable\",\"expr\":\"24\",\"value\":24},\"row\":{\"type\":\"evaluable\",\"expr\":\"4\",\"value\":4},\"address\":{\"type\":\"evaluable\",\"expr\":\"0x0000\",\"value\":0},\"identifier\":\"0\",\"size\":{\"type\":\"evaluable\",\"expr\":\"512\",\"value\":512}},\"equality\":true}]"  deprecateConstraints=0
  FIFO33_2 : aieBasic/FIFO  FifoDepth=512  FIFOType=0  TileType=0  RowLocation=0  ColLocation=0  channel=0  blockJsonConstraints="[{\"type\":\"constraint\",\"constraintType\":\"location_fifo\",\"sid\":\"1167\",\"lhs\":{\"type\":\"location\",\"templParam\":\"fifo\",\"args\":{\"type\":\"fifo\",\"name\":\"DualStreamSSR/SSR8/FIFO33_2\",\"sid\":\"1167\"}},\"rhs\":{\"type\":\"fifogroup\",\"fifotype\":\"dma_fifo\",\"tiletype\":\"aie\",\"column\":{\"type\":\"evaluable\",\"expr\":\"24\",\"value\":24},\"row\":{\"type\":\"evaluable\",\"expr\":\"4\",\"value\":4},\"address\":{\"type\":\"evaluable\",\"expr\":\"0x2000\",\"value\":8192},\"identifier\":\"0\",\"size\":{\"type\":\"evaluable\",\"expr\":\"512\",\"value\":512}},\"equality\":true}]"  deprecateConstraints=0
  FIFO34_1 : aieBasic/FIFO  FifoDepth=512  FIFOType=0  TileType=0  RowLocation=0  ColLocation=0  channel=0  blockJsonConstraints="[{\"type\":\"constraint\",\"constraintType\":\"location_fifo\",\"sid\":\"1191\",\"lhs\":{\"type\":\"location\",\"templParam\":\"fifo\",\"args\":{\"type\":\"fifo\",\"name\":\"DualStreamSSR/SSR8/FIFO34_1\",\"sid\":\"1191\"}},\"rhs\":{\"type\":\"fifogroup\",\"fifotype\":\"dma_fifo\",\"tiletype\":\"aie\",\"column\":{\"type\":\"evaluable\",\"expr\":\"25\",\"value\":25},\"row\":{\"type\":\"evaluable\",\"expr\":\"5\",\"value\":5},\"address\":{\"type\":\"evaluable\",\"expr\":\"0x0000\",\"value\":0},\"identifier\":\"0\",\"size\":{\"type\":\"evaluable\",\"expr\":\"512\",\"value\":512}},\"equality\":true}]"  deprecateConstraints=0
  FIFO34_2 : aieBasic/FIFO  FifoDepth=512  FIFOType=0  TileType=0  RowLocation=0  ColLocation=0  channel=0  blockJsonConstraints="[{\"type\":\"constraint\",\"constraintType\":\"location_fifo\",\"sid\":\"1192\",\"lhs\":{\"type\":\"location\",\"templParam\":\"fifo\",\"args\":{\"type\":\"fifo\",\"name\":\"DualStreamSSR/SSR8/FIFO34_2\",\"sid\":\"1192\"}},\"rhs\":{\"type\":\"fifogroup\",\"fifotype\":\"dma_fifo\",\"tiletype\":\"aie\",\"column\":{\"type\":\"evaluable\",\"expr\":\"25\",\"value\":25},\"row\":{\"type\":\"evaluable\",\"expr\":\"5\",\"value\":5},\"address\":{\"type\":\"evaluable\",\"expr\":\"0x2000\",\"value\":8192},\"identifier\":\"0\",\"size\":{\"type\":\"evaluable\",\"expr\":\"512\",\"value\":512}},\"equality\":true}]"  deprecateConstraints=0
  FIFO35_1 : aieBasic/FIFO  FifoDepth=512  FIFOType=0  TileType=0  RowLocation=0  ColLocation=0  channel=0  blockJsonConstraints="[{\"type\":\"constraint\",\"constraintType\":\"location_fifo\",\"sid\":\"1209\",\"lhs\":{\"type\":\"location\",\"templParam\":\"fifo\",\"args\":{\"type\":\"fifo\",\"name\":\"DualStreamSSR/SSR8/FIFO35_1\",\"sid\":\"1209\"}},\"rhs\":{\"type\":\"fifogroup\",\"fifotype\":\"dma_fifo\",\"tiletype\":\"aie\",\"column\":{\"type\":\"evaluable\",\"expr\":\"26\",\"value\":26},\"row\":{\"type\":\"evaluable\",\"expr\":\"5\",\"value\":5},\"address\":{\"type\":\"evaluable\",\"expr\":\"0x0000\",\"value\":0},\"identifier\":\"0\",\"size\":{\"type\":\"evaluable\",\"expr\":\"512\",\"value\":512}},\"equality\":true}]"  deprecateConstraints=0
  FIFO35_2 : aieBasic/FIFO  FifoDepth=512  FIFOType=0  TileType=0  RowLocation=0  ColLocation=0  channel=0  blockJsonConstraints="[{\"type\":\"constraint\",\"constraintType\":\"location_fifo\",\"sid\":\"1210\",\"lhs\":{\"type\":\"location\",\"templParam\":\"fifo\",\"args\":{\"type\":\"fifo\",\"name\":\"DualStreamSSR/SSR8/FIFO35_2\",\"sid\":\"1210\"}},\"rhs\":{\"type\":\"fifogroup\",\"fifotype\":\"dma_fifo\",\"tiletype\":\"aie\",\"column\":{\"type\":\"evaluable\",\"expr\":\"26\",\"value\":26},\"row\":{\"type\":\"evaluable\",\"expr\":\"5\",\"value\":5},\"address\":{\"type\":\"evaluable\",\"expr\":\"0x2000\",\"value\":8192},\"identifier\":\"0\",\"size\":{\"type\":\"evaluable\",\"expr\":\"512\",\"value\":512}},\"equality\":true}]"  deprecateConstraints=0
  FIFO36_1 : aieBasic/FIFO  FifoDepth=512  FIFOType=0  TileType=0  RowLocation=0  ColLocation=0  channel=0  blockJsonConstraints="[{\"type\":\"constraint\",\"constraintType\":\"location_fifo\",\"sid\":\"1225\",\"lhs\":{\"type\":\"location\",\"templParam\":\"fifo\",\"args\":{\"type\":\"fifo\",\"name\":\"DualStreamSSR/SSR8/FIFO36_1\",\"sid\":\"1225\"}},\"rhs\":{\"type\":\"fifogroup\",\"fifotype\":\"dma_fifo\",\"tiletype\":\"aie\",\"column\":{\"type\":\"evaluable\",\"expr\":\"27\",\"value\":27},\"row\":{\"type\":\"evaluable\",\"expr\":\"5\",\"value\":5},\"address\":{\"type\":\"evaluable\",\"expr\":\"0x0000\",\"value\":0},\"identifier\":\"0\",\"size\":{\"type\":\"evaluable\",\"expr\":\"512\",\"value\":512}},\"equality\":true}]"  deprecateConstraints=0
  FIFO36_2 : aieBasic/FIFO  FifoDepth=512  FIFOType=0  TileType=0  RowLocation=0  ColLocation=0  channel=0  blockJsonConstraints="[{\"type\":\"constraint\",\"constraintType\":\"location_fifo\",\"sid\":\"1226\",\"lhs\":{\"type\":\"location\",\"templParam\":\"fifo\",\"args\":{\"type\":\"fifo\",\"name\":\"DualStreamSSR/SSR8/FIFO36_2\",\"sid\":\"1226\"}},\"rhs\":{\"type\":\"fifogroup\",\"fifotype\":\"dma_fifo\",\"tiletype\":\"aie\",\"column\":{\"type\":\"evaluable\",\"expr\":\"27\",\"value\":27},\"row\":{\"type\":\"evaluable\",\"expr\":\"5\",\"value\":5},\"address\":{\"type\":\"evaluable\",\"expr\":\"0x2000\",\"value\":8192},\"identifier\":\"0\",\"size\":{\"type\":\"evaluable\",\"expr\":\"512\",\"value\":512}},\"equality\":true}]"  deprecateConstraints=0
  FIFO37_1 : aieBasic/FIFO  FifoDepth=512  FIFOType=0  TileType=0  RowLocation=0  ColLocation=0  channel=0  blockJsonConstraints="[{\"type\":\"constraint\",\"constraintType\":\"location_fifo\",\"sid\":\"1241\",\"lhs\":{\"type\":\"location\",\"templParam\":\"fifo\",\"args\":{\"type\":\"fifo\",\"name\":\"DualStreamSSR/SSR8/FIFO37_1\",\"sid\":\"1241\"}},\"rhs\":{\"type\":\"fifogroup\",\"fifotype\":\"dma_fifo\",\"tiletype\":\"aie\",\"column\":{\"type\":\"evaluable\",\"expr\":\"28\",\"value\":28},\"row\":{\"type\":\"evaluable\",\"expr\":\"5\",\"value\":5},\"address\":{\"type\":\"evaluable\",\"expr\":\"0x0000\",\"value\":0},\"identifier\":\"0\",\"size\":{\"type\":\"evaluable\",\"expr\":\"512\",\"value\":512}},\"equality\":true}]"  deprecateConstraints=0
  FIFO37_2 : aieBasic/FIFO  FifoDepth=512  FIFOType=0  TileType=0  RowLocation=0  ColLocation=0  channel=0  blockJsonConstraints="[{\"type\":\"constraint\",\"constraintType\":\"location_fifo\",\"sid\":\"1242\",\"lhs\":{\"type\":\"location\",\"templParam\":\"fifo\",\"args\":{\"type\":\"fifo\",\"name\":\"DualStreamSSR/SSR8/FIFO37_2\",\"sid\":\"1242\"}},\"rhs\":{\"type\":\"fifogroup\",\"fifotype\":\"dma_fifo\",\"tiletype\":\"aie\",\"column\":{\"type\":\"evaluable\",\"expr\":\"28\",\"value\":28},\"row\":{\"type\":\"evaluable\",\"expr\":\"5\",\"value\":5},\"address\":{\"type\":\"evaluable\",\"expr\":\"0x2000\",\"value\":8192},\"identifier\":\"0\",\"size\":{\"type\":\"evaluable\",\"expr\":\"512\",\"value\":512}},\"equality\":true}]"  deprecateConstraints=0
  FIFO38_1 : aieBasic/FIFO  FifoDepth=512  FIFOType=0  TileType=0  RowLocation=0  ColLocation=0  channel=0  blockJsonConstraints="[{\"type\":\"constraint\",\"constraintType\":\"location_fifo\",\"sid\":\"1174\",\"lhs\":{\"type\":\"location\",\"templParam\":\"fifo\",\"args\":{\"type\":\"fifo\",\"name\":\"DualStreamSSR/SSR8/FIFO38_1\",\"sid\":\"1174\"}},\"rhs\":{\"type\":\"fifogroup\",\"fifotype\":\"dma_fifo\",\"tiletype\":\"aie\",\"column\":{\"type\":\"evaluable\",\"expr\":\"24\",\"value\":24},\"row\":{\"type\":\"evaluable\",\"expr\":\"5\",\"value\":5},\"address\":{\"type\":\"evaluable\",\"expr\":\"0x0000\",\"value\":0},\"identifier\":\"0\",\"size\":{\"type\":\"evaluable\",\"expr\":\"512\",\"value\":512}},\"equality\":true}]"  deprecateConstraints=0
  FIFO38_2 : aieBasic/FIFO  FifoDepth=512  FIFOType=0  TileType=0  RowLocation=0  ColLocation=0  channel=0  blockJsonConstraints="[{\"type\":\"constraint\",\"constraintType\":\"location_fifo\",\"sid\":\"1175\",\"lhs\":{\"type\":\"location\",\"templParam\":\"fifo\",\"args\":{\"type\":\"fifo\",\"name\":\"DualStreamSSR/SSR8/FIFO38_2\",\"sid\":\"1175\"}},\"rhs\":{\"type\":\"fifogroup\",\"fifotype\":\"dma_fifo\",\"tiletype\":\"aie\",\"column\":{\"type\":\"evaluable\",\"expr\":\"24\",\"value\":24},\"row\":{\"type\":\"evaluable\",\"expr\":\"5\",\"value\":5},\"address\":{\"type\":\"evaluable\",\"expr\":\"0x2000\",\"value\":8192},\"identifier\":\"0\",\"size\":{\"type\":\"evaluable\",\"expr\":\"512\",\"value\":512}},\"equality\":true}]"  deprecateConstraints=0
  FIFO39_1 : aieBasic/FIFO  FifoDepth=512  FIFOType=0  TileType=0  RowLocation=0  ColLocation=0  channel=0  blockJsonConstraints="[{\"type\":\"constraint\",\"constraintType\":\"location_fifo\",\"sid\":\"1158\",\"lhs\":{\"type\":\"location\",\"templParam\":\"fifo\",\"args\":{\"type\":\"fifo\",\"name\":\"DualStreamSSR/SSR8/FIFO39_1\",\"sid\":\"1158\"}},\"rhs\":{\"type\":\"fifogroup\",\"fifotype\":\"dma_fifo\",\"tiletype\":\"aie\",\"column\":{\"type\":\"evaluable\",\"expr\":\"23\",\"value\":23},\"row\":{\"type\":\"evaluable\",\"expr\":\"5\",\"value\":5},\"address\":{\"type\":\"evaluable\",\"expr\":\"0x0000\",\"value\":0},\"identifier\":\"0\",\"size\":{\"type\":\"evaluable\",\"expr\":\"512\",\"value\":512}},\"equality\":true}]"  deprecateConstraints=0
  FIFO39_2 : aieBasic/FIFO  FifoDepth=512  FIFOType=0  TileType=0  RowLocation=0  ColLocation=0  channel=0  blockJsonConstraints="[{\"type\":\"constraint\",\"constraintType\":\"location_fifo\",\"sid\":\"1159\",\"lhs\":{\"type\":\"location\",\"templParam\":\"fifo\",\"args\":{\"type\":\"fifo\",\"name\":\"DualStreamSSR/SSR8/FIFO39_2\",\"sid\":\"1159\"}},\"rhs\":{\"type\":\"fifogroup\",\"fifotype\":\"dma_fifo\",\"tiletype\":\"aie\",\"column\":{\"type\":\"evaluable\",\"expr\":\"23\",\"value\":23},\"row\":{\"type\":\"evaluable\",\"expr\":\"5\",\"value\":5},\"address\":{\"type\":\"evaluable\",\"expr\":\"0x2000\",\"value\":8192},\"identifier\":\"0\",\"size\":{\"type\":\"evaluable\",\"expr\":\"512\",\"value\":512}},\"equality\":true}]"  deprecateConstraints=0
  FIFO3_1 : aieBasic/FIFO  FifoDepth=512  FIFOType=0  TileType=0  RowLocation=0  ColLocation=0  channel=0  blockJsonConstraints="[{\"type\":\"constraint\",\"constraintType\":\"location_fifo\",\"sid\":\"1205\",\"lhs\":{\"type\":\"location\",\"templParam\":\"fifo\",\"args\":{\"type\":\"fifo\",\"name\":\"DualStreamSSR/SSR8/FIFO3_1\",\"sid\":\"1205\"}},\"rhs\":{\"type\":\"fifogroup\",\"fifotype\":\"dma_fifo\",\"tiletype\":\"aie\",\"column\":{\"type\":\"evaluable\",\"expr\":\"26\",\"value\":26},\"row\":{\"type\":\"evaluable\",\"expr\":\"0\",\"value\":0},\"address\":{\"type\":\"evaluable\",\"expr\":\"0x0000\",\"value\":0},\"identifier\":\"0\",\"size\":{\"type\":\"evaluable\",\"expr\":\"512\",\"value\":512}},\"equality\":true}]"  deprecateConstraints=0
  FIFO3_2 : aieBasic/FIFO  FifoDepth=512  FIFOType=0  TileType=0  RowLocation=0  ColLocation=0  channel=0  blockJsonConstraints="[{\"type\":\"constraint\",\"constraintType\":\"location_fifo\",\"sid\":\"1206\",\"lhs\":{\"type\":\"location\",\"templParam\":\"fifo\",\"args\":{\"type\":\"fifo\",\"name\":\"DualStreamSSR/SSR8/FIFO3_2\",\"sid\":\"1206\"}},\"rhs\":{\"type\":\"fifogroup\",\"fifotype\":\"dma_fifo\",\"tiletype\":\"aie\",\"column\":{\"type\":\"evaluable\",\"expr\":\"26\",\"value\":26},\"row\":{\"type\":\"evaluable\",\"expr\":\"0\",\"value\":0},\"address\":{\"type\":\"evaluable\",\"expr\":\"0x2000\",\"value\":8192},\"identifier\":\"0\",\"size\":{\"type\":\"evaluable\",\"expr\":\"512\",\"value\":512}},\"equality\":true}]"  deprecateConstraints=0
  FIFO40_1 : aieBasic/FIFO  FifoDepth=512  FIFOType=0  TileType=0  RowLocation=0  ColLocation=0  channel=0  blockJsonConstraints="[{\"type\":\"constraint\",\"constraintType\":\"location_fifo\",\"sid\":\"1147\",\"lhs\":{\"type\":\"location\",\"templParam\":\"fifo\",\"args\":{\"type\":\"fifo\",\"name\":\"DualStreamSSR/SSR8/FIFO40_1\",\"sid\":\"1147\"}},\"rhs\":{\"type\":\"fifogroup\",\"fifotype\":\"dma_fifo\",\"tiletype\":\"aie\",\"column\":{\"type\":\"evaluable\",\"expr\":\"23\",\"value\":23},\"row\":{\"type\":\"evaluable\",\"expr\":\"6\",\"value\":6},\"address\":{\"type\":\"evaluable\",\"expr\":\"0x0000\",\"value\":0},\"identifier\":\"0\",\"size\":{\"type\":\"evaluable\",\"expr\":\"512\",\"value\":512}},\"equality\":true}]"  deprecateConstraints=0
  FIFO40_2 : aieBasic/FIFO  FifoDepth=512  FIFOType=0  TileType=0  RowLocation=0  ColLocation=0  channel=0  blockJsonConstraints="[{\"type\":\"constraint\",\"constraintType\":\"location_fifo\",\"sid\":\"1148\",\"lhs\":{\"type\":\"location\",\"templParam\":\"fifo\",\"args\":{\"type\":\"fifo\",\"name\":\"DualStreamSSR/SSR8/FIFO40_2\",\"sid\":\"1148\"}},\"rhs\":{\"type\":\"fifogroup\",\"fifotype\":\"dma_fifo\",\"tiletype\":\"aie\",\"column\":{\"type\":\"evaluable\",\"expr\":\"23\",\"value\":23},\"row\":{\"type\":\"evaluable\",\"expr\":\"6\",\"value\":6},\"address\":{\"type\":\"evaluable\",\"expr\":\"0x2000\",\"value\":8192},\"identifier\":\"0\",\"size\":{\"type\":\"evaluable\",\"expr\":\"512\",\"value\":512}},\"equality\":true}]"  deprecateConstraints=0
  FIFO41_1 : aieBasic/FIFO  FifoDepth=512  FIFOType=0  TileType=0  RowLocation=0  ColLocation=0  channel=0  blockJsonConstraints="[{\"type\":\"constraint\",\"constraintType\":\"location_fifo\",\"sid\":\"1164\",\"lhs\":{\"type\":\"location\",\"templParam\":\"fifo\",\"args\":{\"type\":\"fifo\",\"name\":\"DualStreamSSR/SSR8/FIFO41_1\",\"sid\":\"1164\"}},\"rhs\":{\"type\":\"fifogroup\",\"fifotype\":\"dma_fifo\",\"tiletype\":\"aie\",\"column\":{\"type\":\"evaluable\",\"expr\":\"24\",\"value\":24},\"row\":{\"type\":\"evaluable\",\"expr\":\"6\",\"value\":6},\"address\":{\"type\":\"evaluable\",\"expr\":\"0x0000\",\"value\":0},\"identifier\":\"0\",\"size\":{\"type\":\"evaluable\",\"expr\":\"512\",\"value\":512}},\"equality\":true}]"  deprecateConstraints=0
  FIFO41_2 : aieBasic/FIFO  FifoDepth=512  FIFOType=0  TileType=0  RowLocation=0  ColLocation=0  channel=0  blockJsonConstraints="[{\"type\":\"constraint\",\"constraintType\":\"location_fifo\",\"sid\":\"1165\",\"lhs\":{\"type\":\"location\",\"templParam\":\"fifo\",\"args\":{\"type\":\"fifo\",\"name\":\"DualStreamSSR/SSR8/FIFO41_2\",\"sid\":\"1165\"}},\"rhs\":{\"type\":\"fifogroup\",\"fifotype\":\"dma_fifo\",\"tiletype\":\"aie\",\"column\":{\"type\":\"evaluable\",\"expr\":\"24\",\"value\":24},\"row\":{\"type\":\"evaluable\",\"expr\":\"6\",\"value\":6},\"address\":{\"type\":\"evaluable\",\"expr\":\"0x2000\",\"value\":8192},\"identifier\":\"0\",\"size\":{\"type\":\"evaluable\",\"expr\":\"512\",\"value\":512}},\"equality\":true}]"  deprecateConstraints=0
  FIFO42_1 : aieBasic/FIFO  FifoDepth=512  FIFOType=0  TileType=0  RowLocation=0  ColLocation=0  channel=0  blockJsonConstraints="[{\"type\":\"constraint\",\"constraintType\":\"location_fifo\",\"sid\":\"1207\",\"lhs\":{\"type\":\"location\",\"templParam\":\"fifo\",\"args\":{\"type\":\"fifo\",\"name\":\"DualStreamSSR/SSR8/FIFO42_1\",\"sid\":\"1207\"}},\"rhs\":{\"type\":\"fifogroup\",\"fifotype\":\"dma_fifo\",\"tiletype\":\"aie\",\"column\":{\"type\":\"evaluable\",\"expr\":\"26\",\"value\":26},\"row\":{\"type\":\"evaluable\",\"expr\":\"7\",\"value\":7},\"address\":{\"type\":\"evaluable\",\"expr\":\"0x0000\",\"value\":0},\"identifier\":\"0\",\"size\":{\"type\":\"evaluable\",\"expr\":\"512\",\"value\":512}},\"equality\":true}]"  deprecateConstraints=0
  FIFO42_2 : aieBasic/FIFO  FifoDepth=512  FIFOType=0  TileType=0  RowLocation=0  ColLocation=0  channel=0  blockJsonConstraints="[{\"type\":\"constraint\",\"constraintType\":\"location_fifo\",\"sid\":\"1208\",\"lhs\":{\"type\":\"location\",\"templParam\":\"fifo\",\"args\":{\"type\":\"fifo\",\"name\":\"DualStreamSSR/SSR8/FIFO42_2\",\"sid\":\"1208\"}},\"rhs\":{\"type\":\"fifogroup\",\"fifotype\":\"dma_fifo\",\"tiletype\":\"aie\",\"column\":{\"type\":\"evaluable\",\"expr\":\"26\",\"value\":26},\"row\":{\"type\":\"evaluable\",\"expr\":\"7\",\"value\":7},\"address\":{\"type\":\"evaluable\",\"expr\":\"0x2000\",\"value\":8192},\"identifier\":\"0\",\"size\":{\"type\":\"evaluable\",\"expr\":\"512\",\"value\":512}},\"equality\":true}]"  deprecateConstraints=0
  FIFO43_1 : aieBasic/FIFO  FifoDepth=512  FIFOType=0  TileType=0  RowLocation=0  ColLocation=0  channel=0  blockJsonConstraints="[{\"type\":\"constraint\",\"constraintType\":\"location_fifo\",\"sid\":\"1223\",\"lhs\":{\"type\":\"location\",\"templParam\":\"fifo\",\"args\":{\"type\":\"fifo\",\"name\":\"DualStreamSSR/SSR8/FIFO43_1\",\"sid\":\"1223\"}},\"rhs\":{\"type\":\"fifogroup\",\"fifotype\":\"dma_fifo\",\"tiletype\":\"aie\",\"column\":{\"type\":\"evaluable\",\"expr\":\"27\",\"value\":27},\"row\":{\"type\":\"evaluable\",\"expr\":\"7\",\"value\":7},\"address\":{\"type\":\"evaluable\",\"expr\":\"0x0000\",\"value\":0},\"identifier\":\"0\",\"size\":{\"type\":\"evaluable\",\"expr\":\"512\",\"value\":512}},\"equality\":true}]"  deprecateConstraints=0
  FIFO43_2 : aieBasic/FIFO  FifoDepth=512  FIFOType=0  TileType=0  RowLocation=0  ColLocation=0  channel=0  blockJsonConstraints="[{\"type\":\"constraint\",\"constraintType\":\"location_fifo\",\"sid\":\"1224\",\"lhs\":{\"type\":\"location\",\"templParam\":\"fifo\",\"args\":{\"type\":\"fifo\",\"name\":\"DualStreamSSR/SSR8/FIFO43_2\",\"sid\":\"1224\"}},\"rhs\":{\"type\":\"fifogroup\",\"fifotype\":\"dma_fifo\",\"tiletype\":\"aie\",\"column\":{\"type\":\"evaluable\",\"expr\":\"27\",\"value\":27},\"row\":{\"type\":\"evaluable\",\"expr\":\"7\",\"value\":7},\"address\":{\"type\":\"evaluable\",\"expr\":\"0x2000\",\"value\":8192},\"identifier\":\"0\",\"size\":{\"type\":\"evaluable\",\"expr\":\"512\",\"value\":512}},\"equality\":true}]"  deprecateConstraints=0
  FIFO44_1 : aieBasic/FIFO  FifoDepth=512  FIFOType=0  TileType=0  RowLocation=0  ColLocation=0  channel=0  blockJsonConstraints="[{\"type\":\"constraint\",\"constraintType\":\"location_fifo\",\"sid\":\"1182\",\"lhs\":{\"type\":\"location\",\"templParam\":\"fifo\",\"args\":{\"type\":\"fifo\",\"name\":\"DualStreamSSR/SSR8/FIFO44_1\",\"sid\":\"1182\"}},\"rhs\":{\"type\":\"fifogroup\",\"fifotype\":\"dma_fifo\",\"tiletype\":\"aie\",\"column\":{\"type\":\"evaluable\",\"expr\":\"25\",\"value\":25},\"row\":{\"type\":\"evaluable\",\"expr\":\"4\",\"value\":4},\"address\":{\"type\":\"evaluable\",\"expr\":\"0x0000\",\"value\":0},\"identifier\":\"0\",\"size\":{\"type\":\"evaluable\",\"expr\":\"512\",\"value\":512}},\"equality\":true}]"  deprecateConstraints=0
  FIFO44_2 : aieBasic/FIFO  FifoDepth=512  FIFOType=0  TileType=0  RowLocation=0  ColLocation=0  channel=0  blockJsonConstraints="[{\"type\":\"constraint\",\"constraintType\":\"location_fifo\",\"sid\":\"1183\",\"lhs\":{\"type\":\"location\",\"templParam\":\"fifo\",\"args\":{\"type\":\"fifo\",\"name\":\"DualStreamSSR/SSR8/FIFO44_2\",\"sid\":\"1183\"}},\"rhs\":{\"type\":\"fifogroup\",\"fifotype\":\"dma_fifo\",\"tiletype\":\"aie\",\"column\":{\"type\":\"evaluable\",\"expr\":\"25\",\"value\":25},\"row\":{\"type\":\"evaluable\",\"expr\":\"4\",\"value\":4},\"address\":{\"type\":\"evaluable\",\"expr\":\"0x2000\",\"value\":8192},\"identifier\":\"0\",\"size\":{\"type\":\"evaluable\",\"expr\":\"512\",\"value\":512}},\"equality\":true}]"  deprecateConstraints=0
  FIFO45_1 : aieBasic/FIFO  FifoDepth=512  FIFOType=0  TileType=0  RowLocation=0  ColLocation=0  channel=0  blockJsonConstraints="[{\"type\":\"constraint\",\"constraintType\":\"location_fifo\",\"sid\":\"1239\",\"lhs\":{\"type\":\"location\",\"templParam\":\"fifo\",\"args\":{\"type\":\"fifo\",\"name\":\"DualStreamSSR/SSR8/FIFO45_1\",\"sid\":\"1239\"}},\"rhs\":{\"type\":\"fifogroup\",\"fifotype\":\"dma_fifo\",\"tiletype\":\"aie\",\"column\":{\"type\":\"evaluable\",\"expr\":\"28\",\"value\":28},\"row\":{\"type\":\"evaluable\",\"expr\":\"7\",\"value\":7},\"address\":{\"type\":\"evaluable\",\"expr\":\"0x0000\",\"value\":0},\"identifier\":\"0\",\"size\":{\"type\":\"evaluable\",\"expr\":\"512\",\"value\":512}},\"equality\":true}]"  deprecateConstraints=0
  FIFO45_2 : aieBasic/FIFO  FifoDepth=512  FIFOType=0  TileType=0  RowLocation=0  ColLocation=0  channel=0  blockJsonConstraints="[{\"type\":\"constraint\",\"constraintType\":\"location_fifo\",\"sid\":\"1240\",\"lhs\":{\"type\":\"location\",\"templParam\":\"fifo\",\"args\":{\"type\":\"fifo\",\"name\":\"DualStreamSSR/SSR8/FIFO45_2\",\"sid\":\"1240\"}},\"rhs\":{\"type\":\"fifogroup\",\"fifotype\":\"dma_fifo\",\"tiletype\":\"aie\",\"column\":{\"type\":\"evaluable\",\"expr\":\"28\",\"value\":28},\"row\":{\"type\":\"evaluable\",\"expr\":\"7\",\"value\":7},\"address\":{\"type\":\"evaluable\",\"expr\":\"0x2000\",\"value\":8192},\"identifier\":\"0\",\"size\":{\"type\":\"evaluable\",\"expr\":\"512\",\"value\":512}},\"equality\":true}]"  deprecateConstraints=0
  FIFO46_1 : aieBasic/FIFO  FifoDepth=512  FIFOType=0  TileType=0  RowLocation=0  ColLocation=0  channel=0  blockJsonConstraints="[{\"type\":\"constraint\",\"constraintType\":\"location_fifo\",\"sid\":\"1189\",\"lhs\":{\"type\":\"location\",\"templParam\":\"fifo\",\"args\":{\"type\":\"fifo\",\"name\":\"DualStreamSSR/SSR8/FIFO46_1\",\"sid\":\"1189\"}},\"rhs\":{\"type\":\"fifogroup\",\"fifotype\":\"dma_fifo\",\"tiletype\":\"aie\",\"column\":{\"type\":\"evaluable\",\"expr\":\"25\",\"value\":25},\"row\":{\"type\":\"evaluable\",\"expr\":\"7\",\"value\":7},\"address\":{\"type\":\"evaluable\",\"expr\":\"0x0000\",\"value\":0},\"identifier\":\"0\",\"size\":{\"type\":\"evaluable\",\"expr\":\"512\",\"value\":512}},\"equality\":true}]"  deprecateConstraints=0
  FIFO46_2 : aieBasic/FIFO  FifoDepth=512  FIFOType=0  TileType=0  RowLocation=0  ColLocation=0  channel=0  blockJsonConstraints="[{\"type\":\"constraint\",\"constraintType\":\"location_fifo\",\"sid\":\"1190\",\"lhs\":{\"type\":\"location\",\"templParam\":\"fifo\",\"args\":{\"type\":\"fifo\",\"name\":\"DualStreamSSR/SSR8/FIFO46_2\",\"sid\":\"1190\"}},\"rhs\":{\"type\":\"fifogroup\",\"fifotype\":\"dma_fifo\",\"tiletype\":\"aie\",\"column\":{\"type\":\"evaluable\",\"expr\":\"25\",\"value\":25},\"row\":{\"type\":\"evaluable\",\"expr\":\"7\",\"value\":7},\"address\":{\"type\":\"evaluable\",\"expr\":\"0x2000\",\"value\":8192},\"identifier\":\"0\",\"size\":{\"type\":\"evaluable\",\"expr\":\"512\",\"value\":512}},\"equality\":true}]"  deprecateConstraints=0
  FIFO47_1 : aieBasic/FIFO  FifoDepth=512  FIFOType=0  TileType=0  RowLocation=0  ColLocation=0  channel=0  blockJsonConstraints="[{\"type\":\"constraint\",\"constraintType\":\"location_fifo\",\"sid\":\"1172\",\"lhs\":{\"type\":\"location\",\"templParam\":\"fifo\",\"args\":{\"type\":\"fifo\",\"name\":\"DualStreamSSR/SSR8/FIFO47_1\",\"sid\":\"1172\"}},\"rhs\":{\"type\":\"fifogroup\",\"fifotype\":\"dma_fifo\",\"tiletype\":\"aie\",\"column\":{\"type\":\"evaluable\",\"expr\":\"24\",\"value\":24},\"row\":{\"type\":\"evaluable\",\"expr\":\"7\",\"value\":7},\"address\":{\"type\":\"evaluable\",\"expr\":\"0x0000\",\"value\":0},\"identifier\":\"0\",\"size\":{\"type\":\"evaluable\",\"expr\":\"512\",\"value\":512}},\"equality\":true}]"  deprecateConstraints=0
  FIFO47_2 : aieBasic/FIFO  FifoDepth=512  FIFOType=0  TileType=0  RowLocation=0  ColLocation=0  channel=0  blockJsonConstraints="[{\"type\":\"constraint\",\"constraintType\":\"location_fifo\",\"sid\":\"1173\",\"lhs\":{\"type\":\"location\",\"templParam\":\"fifo\",\"args\":{\"type\":\"fifo\",\"name\":\"DualStreamSSR/SSR8/FIFO47_2\",\"sid\":\"1173\"}},\"rhs\":{\"type\":\"fifogroup\",\"fifotype\":\"dma_fifo\",\"tiletype\":\"aie\",\"column\":{\"type\":\"evaluable\",\"expr\":\"24\",\"value\":24},\"row\":{\"type\":\"evaluable\",\"expr\":\"7\",\"value\":7},\"address\":{\"type\":\"evaluable\",\"expr\":\"0x2000\",\"value\":8192},\"identifier\":\"0\",\"size\":{\"type\":\"evaluable\",\"expr\":\"512\",\"value\":512}},\"equality\":true}]"  deprecateConstraints=0
  FIFO48_1 : aieBasic/FIFO  FifoDepth=512  FIFOType=0  TileType=0  RowLocation=0  ColLocation=0  channel=0  blockJsonConstraints="[{\"type\":\"constraint\",\"constraintType\":\"location_fifo\",\"sid\":\"1155\",\"lhs\":{\"type\":\"location\",\"templParam\":\"fifo\",\"args\":{\"type\":\"fifo\",\"name\":\"DualStreamSSR/SSR8/FIFO48_1\",\"sid\":\"1155\"}},\"rhs\":{\"type\":\"fifogroup\",\"fifotype\":\"dma_fifo\",\"tiletype\":\"aie\",\"column\":{\"type\":\"evaluable\",\"expr\":\"23\",\"value\":23},\"row\":{\"type\":\"evaluable\",\"expr\":\"7\",\"value\":7},\"address\":{\"type\":\"evaluable\",\"expr\":\"0x0000\",\"value\":0},\"identifier\":\"0\",\"size\":{\"type\":\"evaluable\",\"expr\":\"512\",\"value\":512}},\"equality\":true}]"  deprecateConstraints=0
  FIFO48_2 : aieBasic/FIFO  FifoDepth=512  FIFOType=0  TileType=0  RowLocation=0  ColLocation=0  channel=0  blockJsonConstraints="[{\"type\":\"constraint\",\"constraintType\":\"location_fifo\",\"sid\":\"1157\",\"lhs\":{\"type\":\"location\",\"templParam\":\"fifo\",\"args\":{\"type\":\"fifo\",\"name\":\"DualStreamSSR/SSR8/FIFO48_2\",\"sid\":\"1157\"}},\"rhs\":{\"type\":\"fifogroup\",\"fifotype\":\"dma_fifo\",\"tiletype\":\"aie\",\"column\":{\"type\":\"evaluable\",\"expr\":\"23\",\"value\":23},\"row\":{\"type\":\"evaluable\",\"expr\":\"7\",\"value\":7},\"address\":{\"type\":\"evaluable\",\"expr\":\"0x2000\",\"value\":8192},\"identifier\":\"0\",\"size\":{\"type\":\"evaluable\",\"expr\":\"512\",\"value\":512}},\"equality\":true}]"  deprecateConstraints=0
  FIFO49_1 : aieBasic/FIFO  FifoDepth=512  FIFOType=0  TileType=0  RowLocation=0  ColLocation=0  channel=0  blockJsonConstraints="[{\"type\":\"constraint\",\"constraintType\":\"location_fifo\",\"sid\":\"1180\",\"lhs\":{\"type\":\"location\",\"templParam\":\"fifo\",\"args\":{\"type\":\"fifo\",\"name\":\"DualStreamSSR/SSR8/FIFO49_1\",\"sid\":\"1180\"}},\"rhs\":{\"type\":\"fifogroup\",\"fifotype\":\"dma_fifo\",\"tiletype\":\"aie\",\"column\":{\"type\":\"evaluable\",\"expr\":\"25\",\"value\":25},\"row\":{\"type\":\"evaluable\",\"expr\":\"6\",\"value\":6},\"address\":{\"type\":\"evaluable\",\"expr\":\"0x0000\",\"value\":0},\"identifier\":\"0\",\"size\":{\"type\":\"evaluable\",\"expr\":\"512\",\"value\":512}},\"equality\":true}]"  deprecateConstraints=0
  FIFO49_2 : aieBasic/FIFO  FifoDepth=512  FIFOType=0  TileType=0  RowLocation=0  ColLocation=0  channel=0  blockJsonConstraints="[{\"type\":\"constraint\",\"constraintType\":\"location_fifo\",\"sid\":\"1181\",\"lhs\":{\"type\":\"location\",\"templParam\":\"fifo\",\"args\":{\"type\":\"fifo\",\"name\":\"DualStreamSSR/SSR8/FIFO49_2\",\"sid\":\"1181\"}},\"rhs\":{\"type\":\"fifogroup\",\"fifotype\":\"dma_fifo\",\"tiletype\":\"aie\",\"column\":{\"type\":\"evaluable\",\"expr\":\"25\",\"value\":25},\"row\":{\"type\":\"evaluable\",\"expr\":\"6\",\"value\":6},\"address\":{\"type\":\"evaluable\",\"expr\":\"0x2000\",\"value\":8192},\"identifier\":\"0\",\"size\":{\"type\":\"evaluable\",\"expr\":\"512\",\"value\":512}},\"equality\":true}]"  deprecateConstraints=0
  FIFO4_1 : aieBasic/FIFO  FifoDepth=512  FIFOType=0  TileType=0  RowLocation=0  ColLocation=0  channel=0  blockJsonConstraints="[{\"type\":\"constraint\",\"constraintType\":\"location_fifo\",\"sid\":\"1221\",\"lhs\":{\"type\":\"location\",\"templParam\":\"fifo\",\"args\":{\"type\":\"fifo\",\"name\":\"DualStreamSSR/SSR8/FIFO4_1\",\"sid\":\"1221\"}},\"rhs\":{\"type\":\"fifogroup\",\"fifotype\":\"dma_fifo\",\"tiletype\":\"aie\",\"column\":{\"type\":\"evaluable\",\"expr\":\"27\",\"value\":27},\"row\":{\"type\":\"evaluable\",\"expr\":\"0\",\"value\":0},\"address\":{\"type\":\"evaluable\",\"expr\":\"0x0000\",\"value\":0},\"identifier\":\"0\",\"size\":{\"type\":\"evaluable\",\"expr\":\"512\",\"value\":512}},\"equality\":true}]"  deprecateConstraints=0
  FIFO4_2 : aieBasic/FIFO  FifoDepth=512  FIFOType=0  TileType=0  RowLocation=0  ColLocation=0  channel=0  blockJsonConstraints="[{\"type\":\"constraint\",\"constraintType\":\"location_fifo\",\"sid\":\"1222\",\"lhs\":{\"type\":\"location\",\"templParam\":\"fifo\",\"args\":{\"type\":\"fifo\",\"name\":\"DualStreamSSR/SSR8/FIFO4_2\",\"sid\":\"1222\"}},\"rhs\":{\"type\":\"fifogroup\",\"fifotype\":\"dma_fifo\",\"tiletype\":\"aie\",\"column\":{\"type\":\"evaluable\",\"expr\":\"27\",\"value\":27},\"row\":{\"type\":\"evaluable\",\"expr\":\"0\",\"value\":0},\"address\":{\"type\":\"evaluable\",\"expr\":\"0x2000\",\"value\":8192},\"identifier\":\"0\",\"size\":{\"type\":\"evaluable\",\"expr\":\"512\",\"value\":512}},\"equality\":true}]"  deprecateConstraints=0
  FIFO50_1 : aieBasic/FIFO  FifoDepth=512  FIFOType=0  TileType=0  RowLocation=0  ColLocation=0  channel=0  blockJsonConstraints="[{\"type\":\"constraint\",\"constraintType\":\"location_fifo\",\"sid\":\"1199\",\"lhs\":{\"type\":\"location\",\"templParam\":\"fifo\",\"args\":{\"type\":\"fifo\",\"name\":\"DualStreamSSR/SSR8/FIFO50_1\",\"sid\":\"1199\"}},\"rhs\":{\"type\":\"fifogroup\",\"fifotype\":\"dma_fifo\",\"tiletype\":\"aie\",\"column\":{\"type\":\"evaluable\",\"expr\":\"26\",\"value\":26},\"row\":{\"type\":\"evaluable\",\"expr\":\"6\",\"value\":6},\"address\":{\"type\":\"evaluable\",\"expr\":\"0x0000\",\"value\":0},\"identifier\":\"0\",\"size\":{\"type\":\"evaluable\",\"expr\":\"512\",\"value\":512}},\"equality\":true}]"  deprecateConstraints=0
  FIFO50_2 : aieBasic/FIFO  FifoDepth=512  FIFOType=0  TileType=0  RowLocation=0  ColLocation=0  channel=0  blockJsonConstraints="[{\"type\":\"constraint\",\"constraintType\":\"location_fifo\",\"sid\":\"1200\",\"lhs\":{\"type\":\"location\",\"templParam\":\"fifo\",\"args\":{\"type\":\"fifo\",\"name\":\"DualStreamSSR/SSR8/FIFO50_2\",\"sid\":\"1200\"}},\"rhs\":{\"type\":\"fifogroup\",\"fifotype\":\"dma_fifo\",\"tiletype\":\"aie\",\"column\":{\"type\":\"evaluable\",\"expr\":\"26\",\"value\":26},\"row\":{\"type\":\"evaluable\",\"expr\":\"6\",\"value\":6},\"address\":{\"type\":\"evaluable\",\"expr\":\"0x2000\",\"value\":8192},\"identifier\":\"0\",\"size\":{\"type\":\"evaluable\",\"expr\":\"512\",\"value\":512}},\"equality\":true}]"  deprecateConstraints=0
  FIFO51_1 : aieBasic/FIFO  FifoDepth=512  FIFOType=0  TileType=0  RowLocation=0  ColLocation=0  channel=0  blockJsonConstraints="[{\"type\":\"constraint\",\"constraintType\":\"location_fifo\",\"sid\":\"1215\",\"lhs\":{\"type\":\"location\",\"templParam\":\"fifo\",\"args\":{\"type\":\"fifo\",\"name\":\"DualStreamSSR/SSR8/FIFO51_1\",\"sid\":\"1215\"}},\"rhs\":{\"type\":\"fifogroup\",\"fifotype\":\"dma_fifo\",\"tiletype\":\"aie\",\"column\":{\"type\":\"evaluable\",\"expr\":\"27\",\"value\":27},\"row\":{\"type\":\"evaluable\",\"expr\":\"6\",\"value\":6},\"address\":{\"type\":\"evaluable\",\"expr\":\"0x0000\",\"value\":0},\"identifier\":\"0\",\"size\":{\"type\":\"evaluable\",\"expr\":\"512\",\"value\":512}},\"equality\":true}]"  deprecateConstraints=0
  FIFO51_2 : aieBasic/FIFO  FifoDepth=512  FIFOType=0  TileType=0  RowLocation=0  ColLocation=0  channel=0  blockJsonConstraints="[{\"type\":\"constraint\",\"constraintType\":\"location_fifo\",\"sid\":\"1216\",\"lhs\":{\"type\":\"location\",\"templParam\":\"fifo\",\"args\":{\"type\":\"fifo\",\"name\":\"DualStreamSSR/SSR8/FIFO51_2\",\"sid\":\"1216\"}},\"rhs\":{\"type\":\"fifogroup\",\"fifotype\":\"dma_fifo\",\"tiletype\":\"aie\",\"column\":{\"type\":\"evaluable\",\"expr\":\"27\",\"value\":27},\"row\":{\"type\":\"evaluable\",\"expr\":\"6\",\"value\":6},\"address\":{\"type\":\"evaluable\",\"expr\":\"0x2000\",\"value\":8192},\"identifier\":\"0\",\"size\":{\"type\":\"evaluable\",\"expr\":\"512\",\"value\":512}},\"equality\":true}]"  deprecateConstraints=0
  FIFO52_1 : aieBasic/FIFO  FifoDepth=512  FIFOType=0  TileType=0  RowLocation=0  ColLocation=0  channel=0  blockJsonConstraints="[{\"type\":\"constraint\",\"constraintType\":\"location_fifo\",\"sid\":\"1231\",\"lhs\":{\"type\":\"location\",\"templParam\":\"fifo\",\"args\":{\"type\":\"fifo\",\"name\":\"DualStreamSSR/SSR8/FIFO52_1\",\"sid\":\"1231\"}},\"rhs\":{\"type\":\"fifogroup\",\"fifotype\":\"dma_fifo\",\"tiletype\":\"aie\",\"column\":{\"type\":\"evaluable\",\"expr\":\"28\",\"value\":28},\"row\":{\"type\":\"evaluable\",\"expr\":\"6\",\"value\":6},\"address\":{\"type\":\"evaluable\",\"expr\":\"0x0000\",\"value\":0},\"identifier\":\"0\",\"size\":{\"type\":\"evaluable\",\"expr\":\"512\",\"value\":512}},\"equality\":true}]"  deprecateConstraints=0
  FIFO52_2 : aieBasic/FIFO  FifoDepth=512  FIFOType=0  TileType=0  RowLocation=0  ColLocation=0  channel=0  blockJsonConstraints="[{\"type\":\"constraint\",\"constraintType\":\"location_fifo\",\"sid\":\"1232\",\"lhs\":{\"type\":\"location\",\"templParam\":\"fifo\",\"args\":{\"type\":\"fifo\",\"name\":\"DualStreamSSR/SSR8/FIFO52_2\",\"sid\":\"1232\"}},\"rhs\":{\"type\":\"fifogroup\",\"fifotype\":\"dma_fifo\",\"tiletype\":\"aie\",\"column\":{\"type\":\"evaluable\",\"expr\":\"28\",\"value\":28},\"row\":{\"type\":\"evaluable\",\"expr\":\"6\",\"value\":6},\"address\":{\"type\":\"evaluable\",\"expr\":\"0x2000\",\"value\":8192},\"identifier\":\"0\",\"size\":{\"type\":\"evaluable\",\"expr\":\"512\",\"value\":512}},\"equality\":true}]"  deprecateConstraints=0
  FIFO53_1 : aieBasic/FIFO  FifoDepth=512  FIFOType=0  TileType=0  RowLocation=0  ColLocation=0  channel=0  blockJsonConstraints="[{\"type\":\"constraint\",\"constraintType\":\"location_fifo\",\"sid\":\"1247\",\"lhs\":{\"type\":\"location\",\"templParam\":\"fifo\",\"args\":{\"type\":\"fifo\",\"name\":\"DualStreamSSR/SSR8/FIFO53_1\",\"sid\":\"1247\"}},\"rhs\":{\"type\":\"fifogroup\",\"fifotype\":\"dma_fifo\",\"tiletype\":\"aie\",\"column\":{\"type\":\"evaluable\",\"expr\":\"29\",\"value\":29},\"row\":{\"type\":\"evaluable\",\"expr\":\"6\",\"value\":6},\"address\":{\"type\":\"evaluable\",\"expr\":\"0x0000\",\"value\":0},\"identifier\":\"0\",\"size\":{\"type\":\"evaluable\",\"expr\":\"512\",\"value\":512}},\"equality\":true}]"  deprecateConstraints=0
  FIFO53_2 : aieBasic/FIFO  FifoDepth=512  FIFOType=0  TileType=0  RowLocation=0  ColLocation=0  channel=0  blockJsonConstraints="[{\"type\":\"constraint\",\"constraintType\":\"location_fifo\",\"sid\":\"1248\",\"lhs\":{\"type\":\"location\",\"templParam\":\"fifo\",\"args\":{\"type\":\"fifo\",\"name\":\"DualStreamSSR/SSR8/FIFO53_2\",\"sid\":\"1248\"}},\"rhs\":{\"type\":\"fifogroup\",\"fifotype\":\"dma_fifo\",\"tiletype\":\"aie\",\"column\":{\"type\":\"evaluable\",\"expr\":\"29\",\"value\":29},\"row\":{\"type\":\"evaluable\",\"expr\":\"6\",\"value\":6},\"address\":{\"type\":\"evaluable\",\"expr\":\"0x2000\",\"value\":8192},\"identifier\":\"0\",\"size\":{\"type\":\"evaluable\",\"expr\":\"512\",\"value\":512}},\"equality\":true}]"  deprecateConstraints=0
  FIFO54_1 : aieBasic/FIFO  FifoDepth=512  FIFOType=0  TileType=0  RowLocation=0  ColLocation=0  channel=0  blockJsonConstraints="[{\"type\":\"constraint\",\"constraintType\":\"location_fifo\",\"sid\":\"1263\",\"lhs\":{\"type\":\"location\",\"templParam\":\"fifo\",\"args\":{\"type\":\"fifo\",\"name\":\"DualStreamSSR/SSR8/FIFO54_1\",\"sid\":\"1263\"}},\"rhs\":{\"type\":\"fifogroup\",\"fifotype\":\"dma_fifo\",\"tiletype\":\"aie\",\"column\":{\"type\":\"evaluable\",\"expr\":\"30\",\"value\":30},\"row\":{\"type\":\"evaluable\",\"expr\":\"6\",\"value\":6},\"address\":{\"type\":\"evaluable\",\"expr\":\"0x0000\",\"value\":0},\"identifier\":\"0\",\"size\":{\"type\":\"evaluable\",\"expr\":\"512\",\"value\":512}},\"equality\":true}]"  deprecateConstraints=0
  FIFO54_2 : aieBasic/FIFO  FifoDepth=512  FIFOType=0  TileType=0  RowLocation=0  ColLocation=0  channel=0  blockJsonConstraints="[{\"type\":\"constraint\",\"constraintType\":\"location_fifo\",\"sid\":\"1264\",\"lhs\":{\"type\":\"location\",\"templParam\":\"fifo\",\"args\":{\"type\":\"fifo\",\"name\":\"DualStreamSSR/SSR8/FIFO54_2\",\"sid\":\"1264\"}},\"rhs\":{\"type\":\"fifogroup\",\"fifotype\":\"dma_fifo\",\"tiletype\":\"aie\",\"column\":{\"type\":\"evaluable\",\"expr\":\"30\",\"value\":30},\"row\":{\"type\":\"evaluable\",\"expr\":\"6\",\"value\":6},\"address\":{\"type\":\"evaluable\",\"expr\":\"0x2000\",\"value\":8192},\"identifier\":\"0\",\"size\":{\"type\":\"evaluable\",\"expr\":\"512\",\"value\":512}},\"equality\":true}]"  deprecateConstraints=0
  FIFO55_1 : aieBasic/FIFO  FifoDepth=512  FIFOType=0  TileType=0  RowLocation=0  ColLocation=0  channel=0  blockJsonConstraints="[{\"type\":\"constraint\",\"constraintType\":\"location_fifo\",\"sid\":\"1201\",\"lhs\":{\"type\":\"location\",\"templParam\":\"fifo\",\"args\":{\"type\":\"fifo\",\"name\":\"DualStreamSSR/SSR8/FIFO55_1\",\"sid\":\"1201\"}},\"rhs\":{\"type\":\"fifogroup\",\"fifotype\":\"dma_fifo\",\"tiletype\":\"aie\",\"column\":{\"type\":\"evaluable\",\"expr\":\"26\",\"value\":26},\"row\":{\"type\":\"evaluable\",\"expr\":\"4\",\"value\":4},\"address\":{\"type\":\"evaluable\",\"expr\":\"0x0000\",\"value\":0},\"identifier\":\"0\",\"size\":{\"type\":\"evaluable\",\"expr\":\"512\",\"value\":512}},\"equality\":true}]"  deprecateConstraints=0
  FIFO55_2 : aieBasic/FIFO  FifoDepth=512  FIFOType=0  TileType=0  RowLocation=0  ColLocation=0  channel=0  blockJsonConstraints="[{\"type\":\"constraint\",\"constraintType\":\"location_fifo\",\"sid\":\"1202\",\"lhs\":{\"type\":\"location\",\"templParam\":\"fifo\",\"args\":{\"type\":\"fifo\",\"name\":\"DualStreamSSR/SSR8/FIFO55_2\",\"sid\":\"1202\"}},\"rhs\":{\"type\":\"fifogroup\",\"fifotype\":\"dma_fifo\",\"tiletype\":\"aie\",\"column\":{\"type\":\"evaluable\",\"expr\":\"26\",\"value\":26},\"row\":{\"type\":\"evaluable\",\"expr\":\"4\",\"value\":4},\"address\":{\"type\":\"evaluable\",\"expr\":\"0x2000\",\"value\":8192},\"identifier\":\"0\",\"size\":{\"type\":\"evaluable\",\"expr\":\"512\",\"value\":512}},\"equality\":true}]"  deprecateConstraints=0
  FIFO56_1 : aieBasic/FIFO  FifoDepth=512  FIFOType=0  TileType=0  RowLocation=0  ColLocation=0  channel=0  blockJsonConstraints="[{\"type\":\"constraint\",\"constraintType\":\"location_fifo\",\"sid\":\"1271\",\"lhs\":{\"type\":\"location\",\"templParam\":\"fifo\",\"args\":{\"type\":\"fifo\",\"name\":\"DualStreamSSR/SSR8/FIFO56_1\",\"sid\":\"1271\"}},\"rhs\":{\"type\":\"fifogroup\",\"fifotype\":\"dma_fifo\",\"tiletype\":\"aie\",\"column\":{\"type\":\"evaluable\",\"expr\":\"30\",\"value\":30},\"row\":{\"type\":\"evaluable\",\"expr\":\"7\",\"value\":7},\"address\":{\"type\":\"evaluable\",\"expr\":\"0x0000\",\"value\":0},\"identifier\":\"0\",\"size\":{\"type\":\"evaluable\",\"expr\":\"512\",\"value\":512}},\"equality\":true}]"  deprecateConstraints=0
  FIFO56_2 : aieBasic/FIFO  FifoDepth=512  FIFOType=0  TileType=0  RowLocation=0  ColLocation=0  channel=0  blockJsonConstraints="[{\"type\":\"constraint\",\"constraintType\":\"location_fifo\",\"sid\":\"1272\",\"lhs\":{\"type\":\"location\",\"templParam\":\"fifo\",\"args\":{\"type\":\"fifo\",\"name\":\"DualStreamSSR/SSR8/FIFO56_2\",\"sid\":\"1272\"}},\"rhs\":{\"type\":\"fifogroup\",\"fifotype\":\"dma_fifo\",\"tiletype\":\"aie\",\"column\":{\"type\":\"evaluable\",\"expr\":\"30\",\"value\":30},\"row\":{\"type\":\"evaluable\",\"expr\":\"7\",\"value\":7},\"address\":{\"type\":\"evaluable\",\"expr\":\"0x2000\",\"value\":8192},\"identifier\":\"0\",\"size\":{\"type\":\"evaluable\",\"expr\":\"512\",\"value\":512}},\"equality\":true}]"  deprecateConstraints=0
  FIFO57_1 : aieBasic/FIFO  FifoDepth=512  FIFOType=0  TileType=0  RowLocation=0  ColLocation=0  channel=0  blockJsonConstraints="[{\"type\":\"constraint\",\"constraintType\":\"location_fifo\",\"sid\":\"1255\",\"lhs\":{\"type\":\"location\",\"templParam\":\"fifo\",\"args\":{\"type\":\"fifo\",\"name\":\"DualStreamSSR/SSR8/FIFO57_1\",\"sid\":\"1255\"}},\"rhs\":{\"type\":\"fifogroup\",\"fifotype\":\"dma_fifo\",\"tiletype\":\"aie\",\"column\":{\"type\":\"evaluable\",\"expr\":\"29\",\"value\":29},\"row\":{\"type\":\"evaluable\",\"expr\":\"7\",\"value\":7},\"address\":{\"type\":\"evaluable\",\"expr\":\"0x0000\",\"value\":0},\"identifier\":\"0\",\"size\":{\"type\":\"evaluable\",\"expr\":\"512\",\"value\":512}},\"equality\":true}]"  deprecateConstraints=0
  FIFO57_2 : aieBasic/FIFO  FifoDepth=512  FIFOType=0  TileType=0  RowLocation=0  ColLocation=0  channel=0  blockJsonConstraints="[{\"type\":\"constraint\",\"constraintType\":\"location_fifo\",\"sid\":\"1256\",\"lhs\":{\"type\":\"location\",\"templParam\":\"fifo\",\"args\":{\"type\":\"fifo\",\"name\":\"DualStreamSSR/SSR8/FIFO57_2\",\"sid\":\"1256\"}},\"rhs\":{\"type\":\"fifogroup\",\"fifotype\":\"dma_fifo\",\"tiletype\":\"aie\",\"column\":{\"type\":\"evaluable\",\"expr\":\"29\",\"value\":29},\"row\":{\"type\":\"evaluable\",\"expr\":\"7\",\"value\":7},\"address\":{\"type\":\"evaluable\",\"expr\":\"0x2000\",\"value\":8192},\"identifier\":\"0\",\"size\":{\"type\":\"evaluable\",\"expr\":\"512\",\"value\":512}},\"equality\":true}]"  deprecateConstraints=0
  FIFO58_1 : aieBasic/FIFO  FifoDepth=512  FIFOType=0  TileType=0  RowLocation=0  ColLocation=0  channel=0  blockJsonConstraints="[{\"type\":\"constraint\",\"constraintType\":\"location_fifo\",\"sid\":\"1217\",\"lhs\":{\"type\":\"location\",\"templParam\":\"fifo\",\"args\":{\"type\":\"fifo\",\"name\":\"DualStreamSSR/SSR8/FIFO58_1\",\"sid\":\"1217\"}},\"rhs\":{\"type\":\"fifogroup\",\"fifotype\":\"dma_fifo\",\"tiletype\":\"aie\",\"column\":{\"type\":\"evaluable\",\"expr\":\"27\",\"value\":27},\"row\":{\"type\":\"evaluable\",\"expr\":\"4\",\"value\":4},\"address\":{\"type\":\"evaluable\",\"expr\":\"0x0000\",\"value\":0},\"identifier\":\"0\",\"size\":{\"type\":\"evaluable\",\"expr\":\"512\",\"value\":512}},\"equality\":true}]"  deprecateConstraints=0
  FIFO58_2 : aieBasic/FIFO  FifoDepth=512  FIFOType=0  TileType=0  RowLocation=0  ColLocation=0  channel=0  blockJsonConstraints="[{\"type\":\"constraint\",\"constraintType\":\"location_fifo\",\"sid\":\"1218\",\"lhs\":{\"type\":\"location\",\"templParam\":\"fifo\",\"args\":{\"type\":\"fifo\",\"name\":\"DualStreamSSR/SSR8/FIFO58_2\",\"sid\":\"1218\"}},\"rhs\":{\"type\":\"fifogroup\",\"fifotype\":\"dma_fifo\",\"tiletype\":\"aie\",\"column\":{\"type\":\"evaluable\",\"expr\":\"27\",\"value\":27},\"row\":{\"type\":\"evaluable\",\"expr\":\"4\",\"value\":4},\"address\":{\"type\":\"evaluable\",\"expr\":\"0x2000\",\"value\":8192},\"identifier\":\"0\",\"size\":{\"type\":\"evaluable\",\"expr\":\"512\",\"value\":512}},\"equality\":true}]"  deprecateConstraints=0
  FIFO59_1 : aieBasic/FIFO  FifoDepth=512  FIFOType=0  TileType=0  RowLocation=0  ColLocation=0  channel=0  blockJsonConstraints="[{\"type\":\"constraint\",\"constraintType\":\"location_fifo\",\"sid\":\"1233\",\"lhs\":{\"type\":\"location\",\"templParam\":\"fifo\",\"args\":{\"type\":\"fifo\",\"name\":\"DualStreamSSR/SSR8/FIFO59_1\",\"sid\":\"1233\"}},\"rhs\":{\"type\":\"fifogroup\",\"fifotype\":\"dma_fifo\",\"tiletype\":\"aie\",\"column\":{\"type\":\"evaluable\",\"expr\":\"28\",\"value\":28},\"row\":{\"type\":\"evaluable\",\"expr\":\"4\",\"value\":4},\"address\":{\"type\":\"evaluable\",\"expr\":\"0x0000\",\"value\":0},\"identifier\":\"0\",\"size\":{\"type\":\"evaluable\",\"expr\":\"512\",\"value\":512}},\"equality\":true}]"  deprecateConstraints=0
  FIFO59_2 : aieBasic/FIFO  FifoDepth=512  FIFOType=0  TileType=0  RowLocation=0  ColLocation=0  channel=0  blockJsonConstraints="[{\"type\":\"constraint\",\"constraintType\":\"location_fifo\",\"sid\":\"1234\",\"lhs\":{\"type\":\"location\",\"templParam\":\"fifo\",\"args\":{\"type\":\"fifo\",\"name\":\"DualStreamSSR/SSR8/FIFO59_2\",\"sid\":\"1234\"}},\"rhs\":{\"type\":\"fifogroup\",\"fifotype\":\"dma_fifo\",\"tiletype\":\"aie\",\"column\":{\"type\":\"evaluable\",\"expr\":\"28\",\"value\":28},\"row\":{\"type\":\"evaluable\",\"expr\":\"4\",\"value\":4},\"address\":{\"type\":\"evaluable\",\"expr\":\"0x2000\",\"value\":8192},\"identifier\":\"0\",\"size\":{\"type\":\"evaluable\",\"expr\":\"512\",\"value\":512}},\"equality\":true}]"  deprecateConstraints=0
  FIFO5_1 : aieBasic/FIFO  FifoDepth=512  FIFOType=0  TileType=0  RowLocation=0  ColLocation=0  channel=0  blockJsonConstraints="[{\"type\":\"constraint\",\"constraintType\":\"location_fifo\",\"sid\":\"1237\",\"lhs\":{\"type\":\"location\",\"templParam\":\"fifo\",\"args\":{\"type\":\"fifo\",\"name\":\"DualStreamSSR/SSR8/FIFO5_1\",\"sid\":\"1237\"}},\"rhs\":{\"type\":\"fifogroup\",\"fifotype\":\"dma_fifo\",\"tiletype\":\"aie\",\"column\":{\"type\":\"evaluable\",\"expr\":\"28\",\"value\":28},\"row\":{\"type\":\"evaluable\",\"expr\":\"0\",\"value\":0},\"address\":{\"type\":\"evaluable\",\"expr\":\"0x0000\",\"value\":0},\"identifier\":\"0\",\"size\":{\"type\":\"evaluable\",\"expr\":\"512\",\"value\":512}},\"equality\":true}]"  deprecateConstraints=0
  FIFO5_2 : aieBasic/FIFO  FifoDepth=512  FIFOType=0  TileType=0  RowLocation=0  ColLocation=0  channel=0  blockJsonConstraints="[{\"type\":\"constraint\",\"constraintType\":\"location_fifo\",\"sid\":\"1238\",\"lhs\":{\"type\":\"location\",\"templParam\":\"fifo\",\"args\":{\"type\":\"fifo\",\"name\":\"DualStreamSSR/SSR8/FIFO5_2\",\"sid\":\"1238\"}},\"rhs\":{\"type\":\"fifogroup\",\"fifotype\":\"dma_fifo\",\"tiletype\":\"aie\",\"column\":{\"type\":\"evaluable\",\"expr\":\"28\",\"value\":28},\"row\":{\"type\":\"evaluable\",\"expr\":\"0\",\"value\":0},\"address\":{\"type\":\"evaluable\",\"expr\":\"0x2000\",\"value\":8192},\"identifier\":\"0\",\"size\":{\"type\":\"evaluable\",\"expr\":\"512\",\"value\":512}},\"equality\":true}]"  deprecateConstraints=0
  FIFO60_1 : aieBasic/FIFO  FifoDepth=512  FIFOType=0  TileType=0  RowLocation=0  ColLocation=0  channel=0  blockJsonConstraints="[{\"type\":\"constraint\",\"constraintType\":\"location_fifo\",\"sid\":\"1249\",\"lhs\":{\"type\":\"location\",\"templParam\":\"fifo\",\"args\":{\"type\":\"fifo\",\"name\":\"DualStreamSSR/SSR8/FIFO60_1\",\"sid\":\"1249\"}},\"rhs\":{\"type\":\"fifogroup\",\"fifotype\":\"dma_fifo\",\"tiletype\":\"aie\",\"column\":{\"type\":\"evaluable\",\"expr\":\"29\",\"value\":29},\"row\":{\"type\":\"evaluable\",\"expr\":\"4\",\"value\":4},\"address\":{\"type\":\"evaluable\",\"expr\":\"0x0000\",\"value\":0},\"identifier\":\"0\",\"size\":{\"type\":\"evaluable\",\"expr\":\"512\",\"value\":512}},\"equality\":true}]"  deprecateConstraints=0
  FIFO60_2 : aieBasic/FIFO  FifoDepth=512  FIFOType=0  TileType=0  RowLocation=0  ColLocation=0  channel=0  blockJsonConstraints="[{\"type\":\"constraint\",\"constraintType\":\"location_fifo\",\"sid\":\"1250\",\"lhs\":{\"type\":\"location\",\"templParam\":\"fifo\",\"args\":{\"type\":\"fifo\",\"name\":\"DualStreamSSR/SSR8/FIFO60_2\",\"sid\":\"1250\"}},\"rhs\":{\"type\":\"fifogroup\",\"fifotype\":\"dma_fifo\",\"tiletype\":\"aie\",\"column\":{\"type\":\"evaluable\",\"expr\":\"29\",\"value\":29},\"row\":{\"type\":\"evaluable\",\"expr\":\"4\",\"value\":4},\"address\":{\"type\":\"evaluable\",\"expr\":\"0x2000\",\"value\":8192},\"identifier\":\"0\",\"size\":{\"type\":\"evaluable\",\"expr\":\"512\",\"value\":512}},\"equality\":true}]"  deprecateConstraints=0
  FIFO61_1 : aieBasic/FIFO  FifoDepth=512  FIFOType=0  TileType=0  RowLocation=0  ColLocation=0  channel=0  blockJsonConstraints="[{\"type\":\"constraint\",\"constraintType\":\"location_fifo\",\"sid\":\"1265\",\"lhs\":{\"type\":\"location\",\"templParam\":\"fifo\",\"args\":{\"type\":\"fifo\",\"name\":\"DualStreamSSR/SSR8/FIFO61_1\",\"sid\":\"1265\"}},\"rhs\":{\"type\":\"fifogroup\",\"fifotype\":\"dma_fifo\",\"tiletype\":\"aie\",\"column\":{\"type\":\"evaluable\",\"expr\":\"30\",\"value\":30},\"row\":{\"type\":\"evaluable\",\"expr\":\"4\",\"value\":4},\"address\":{\"type\":\"evaluable\",\"expr\":\"0x0000\",\"value\":0},\"identifier\":\"0\",\"size\":{\"type\":\"evaluable\",\"expr\":\"512\",\"value\":512}},\"equality\":true}]"  deprecateConstraints=0
  FIFO61_2 : aieBasic/FIFO  FifoDepth=512  FIFOType=0  TileType=0  RowLocation=0  ColLocation=0  channel=0  blockJsonConstraints="[{\"type\":\"constraint\",\"constraintType\":\"location_fifo\",\"sid\":\"1266\",\"lhs\":{\"type\":\"location\",\"templParam\":\"fifo\",\"args\":{\"type\":\"fifo\",\"name\":\"DualStreamSSR/SSR8/FIFO61_2\",\"sid\":\"1266\"}},\"rhs\":{\"type\":\"fifogroup\",\"fifotype\":\"dma_fifo\",\"tiletype\":\"aie\",\"column\":{\"type\":\"evaluable\",\"expr\":\"30\",\"value\":30},\"row\":{\"type\":\"evaluable\",\"expr\":\"4\",\"value\":4},\"address\":{\"type\":\"evaluable\",\"expr\":\"0x2000\",\"value\":8192},\"identifier\":\"0\",\"size\":{\"type\":\"evaluable\",\"expr\":\"512\",\"value\":512}},\"equality\":true}]"  deprecateConstraints=0
  FIFO62_1 : aieBasic/FIFO  FifoDepth=512  FIFOType=0  TileType=0  RowLocation=0  ColLocation=0  channel=0  blockJsonConstraints="[{\"type\":\"constraint\",\"constraintType\":\"location_fifo\",\"sid\":\"1273\",\"lhs\":{\"type\":\"location\",\"templParam\":\"fifo\",\"args\":{\"type\":\"fifo\",\"name\":\"DualStreamSSR/SSR8/FIFO62_1\",\"sid\":\"1273\"}},\"rhs\":{\"type\":\"fifogroup\",\"fifotype\":\"dma_fifo\",\"tiletype\":\"aie\",\"column\":{\"type\":\"evaluable\",\"expr\":\"30\",\"value\":30},\"row\":{\"type\":\"evaluable\",\"expr\":\"5\",\"value\":5},\"address\":{\"type\":\"evaluable\",\"expr\":\"0x0000\",\"value\":0},\"identifier\":\"0\",\"size\":{\"type\":\"evaluable\",\"expr\":\"512\",\"value\":512}},\"equality\":true}]"  deprecateConstraints=0
  FIFO62_2 : aieBasic/FIFO  FifoDepth=512  FIFOType=0  TileType=0  RowLocation=0  ColLocation=0  channel=0  blockJsonConstraints="[{\"type\":\"constraint\",\"constraintType\":\"location_fifo\",\"sid\":\"1274\",\"lhs\":{\"type\":\"location\",\"templParam\":\"fifo\",\"args\":{\"type\":\"fifo\",\"name\":\"DualStreamSSR/SSR8/FIFO62_2\",\"sid\":\"1274\"}},\"rhs\":{\"type\":\"fifogroup\",\"fifotype\":\"dma_fifo\",\"tiletype\":\"aie\",\"column\":{\"type\":\"evaluable\",\"expr\":\"30\",\"value\":30},\"row\":{\"type\":\"evaluable\",\"expr\":\"5\",\"value\":5},\"address\":{\"type\":\"evaluable\",\"expr\":\"0x2000\",\"value\":8192},\"identifier\":\"0\",\"size\":{\"type\":\"evaluable\",\"expr\":\"512\",\"value\":512}},\"equality\":true}]"  deprecateConstraints=0
  FIFO63_1 : aieBasic/FIFO  FifoDepth=512  FIFOType=0  TileType=0  RowLocation=0  ColLocation=0  channel=0  blockJsonConstraints="[{\"type\":\"constraint\",\"constraintType\":\"location_fifo\",\"sid\":\"1257\",\"lhs\":{\"type\":\"location\",\"templParam\":\"fifo\",\"args\":{\"type\":\"fifo\",\"name\":\"DualStreamSSR/SSR8/FIFO63_1\",\"sid\":\"1257\"}},\"rhs\":{\"type\":\"fifogroup\",\"fifotype\":\"dma_fifo\",\"tiletype\":\"aie\",\"column\":{\"type\":\"evaluable\",\"expr\":\"29\",\"value\":29},\"row\":{\"type\":\"evaluable\",\"expr\":\"5\",\"value\":5},\"address\":{\"type\":\"evaluable\",\"expr\":\"0x0000\",\"value\":0},\"identifier\":\"0\",\"size\":{\"type\":\"evaluable\",\"expr\":\"512\",\"value\":512}},\"equality\":true}]"  deprecateConstraints=0
  FIFO63_2 : aieBasic/FIFO  FifoDepth=512  FIFOType=0  TileType=0  RowLocation=0  ColLocation=0  channel=0  blockJsonConstraints="[{\"type\":\"constraint\",\"constraintType\":\"location_fifo\",\"sid\":\"1258\",\"lhs\":{\"type\":\"location\",\"templParam\":\"fifo\",\"args\":{\"type\":\"fifo\",\"name\":\"DualStreamSSR/SSR8/FIFO63_2\",\"sid\":\"1258\"}},\"rhs\":{\"type\":\"fifogroup\",\"fifotype\":\"dma_fifo\",\"tiletype\":\"aie\",\"column\":{\"type\":\"evaluable\",\"expr\":\"29\",\"value\":29},\"row\":{\"type\":\"evaluable\",\"expr\":\"5\",\"value\":5},\"address\":{\"type\":\"evaluable\",\"expr\":\"0x2000\",\"value\":8192},\"identifier\":\"0\",\"size\":{\"type\":\"evaluable\",\"expr\":\"512\",\"value\":512}},\"equality\":true}]"  deprecateConstraints=0
  FIFO6_1 : aieBasic/FIFO  FifoDepth=512  FIFOType=0  TileType=0  RowLocation=0  ColLocation=0  channel=0  blockJsonConstraints="[{\"type\":\"constraint\",\"constraintType\":\"location_fifo\",\"sid\":\"1253\",\"lhs\":{\"type\":\"location\",\"templParam\":\"fifo\",\"args\":{\"type\":\"fifo\",\"name\":\"DualStreamSSR/SSR8/FIFO6_1\",\"sid\":\"1253\"}},\"rhs\":{\"type\":\"fifogroup\",\"fifotype\":\"dma_fifo\",\"tiletype\":\"aie\",\"column\":{\"type\":\"evaluable\",\"expr\":\"29\",\"value\":29},\"row\":{\"type\":\"evaluable\",\"expr\":\"0\",\"value\":0},\"address\":{\"type\":\"evaluable\",\"expr\":\"0x0000\",\"value\":0},\"identifier\":\"0\",\"size\":{\"type\":\"evaluable\",\"expr\":\"512\",\"value\":512}},\"equality\":true}]"  deprecateConstraints=0
  FIFO6_2 : aieBasic/FIFO  FifoDepth=512  FIFOType=0  TileType=0  RowLocation=0  ColLocation=0  channel=0  blockJsonConstraints="[{\"type\":\"constraint\",\"constraintType\":\"location_fifo\",\"sid\":\"1254\",\"lhs\":{\"type\":\"location\",\"templParam\":\"fifo\",\"args\":{\"type\":\"fifo\",\"name\":\"DualStreamSSR/SSR8/FIFO6_2\",\"sid\":\"1254\"}},\"rhs\":{\"type\":\"fifogroup\",\"fifotype\":\"dma_fifo\",\"tiletype\":\"aie\",\"column\":{\"type\":\"evaluable\",\"expr\":\"29\",\"value\":29},\"row\":{\"type\":\"evaluable\",\"expr\":\"0\",\"value\":0},\"address\":{\"type\":\"evaluable\",\"expr\":\"0x2000\",\"value\":8192},\"identifier\":\"0\",\"size\":{\"type\":\"evaluable\",\"expr\":\"512\",\"value\":512}},\"equality\":true}]"  deprecateConstraints=0
  FIFO7_1 : aieBasic/FIFO  FifoDepth=512  FIFOType=0  TileType=0  RowLocation=0  ColLocation=0  channel=0  blockJsonConstraints="[{\"type\":\"constraint\",\"constraintType\":\"location_fifo\",\"sid\":\"1269\",\"lhs\":{\"type\":\"location\",\"templParam\":\"fifo\",\"args\":{\"type\":\"fifo\",\"name\":\"DualStreamSSR/SSR8/FIFO7_1\",\"sid\":\"1269\"}},\"rhs\":{\"type\":\"fifogroup\",\"fifotype\":\"dma_fifo\",\"tiletype\":\"aie\",\"column\":{\"type\":\"evaluable\",\"expr\":\"30\",\"value\":30},\"row\":{\"type\":\"evaluable\",\"expr\":\"0\",\"value\":0},\"address\":{\"type\":\"evaluable\",\"expr\":\"0x0000\",\"value\":0},\"identifier\":\"0\",\"size\":{\"type\":\"evaluable\",\"expr\":\"512\",\"value\":512}},\"equality\":true}]"  deprecateConstraints=0
  FIFO7_2 : aieBasic/FIFO  FifoDepth=512  FIFOType=0  TileType=0  RowLocation=0  ColLocation=0  channel=0  blockJsonConstraints="[{\"type\":\"constraint\",\"constraintType\":\"location_fifo\",\"sid\":\"1270\",\"lhs\":{\"type\":\"location\",\"templParam\":\"fifo\",\"args\":{\"type\":\"fifo\",\"name\":\"DualStreamSSR/SSR8/FIFO7_2\",\"sid\":\"1270\"}},\"rhs\":{\"type\":\"fifogroup\",\"fifotype\":\"dma_fifo\",\"tiletype\":\"aie\",\"column\":{\"type\":\"evaluable\",\"expr\":\"30\",\"value\":30},\"row\":{\"type\":\"evaluable\",\"expr\":\"0\",\"value\":0},\"address\":{\"type\":\"evaluable\",\"expr\":\"0x2000\",\"value\":8192},\"identifier\":\"0\",\"size\":{\"type\":\"evaluable\",\"expr\":\"512\",\"value\":512}},\"equality\":true}]"  deprecateConstraints=0
  FIFO8_1 : aieBasic/FIFO  FifoDepth=512  FIFOType=0  TileType=0  RowLocation=0  ColLocation=0  channel=0  blockJsonConstraints="[{\"type\":\"constraint\",\"constraintType\":\"location_fifo\",\"sid\":\"1277\",\"lhs\":{\"type\":\"location\",\"templParam\":\"fifo\",\"args\":{\"type\":\"fifo\",\"name\":\"DualStreamSSR/SSR8/FIFO8_1\",\"sid\":\"1277\"}},\"rhs\":{\"type\":\"fifogroup\",\"fifotype\":\"dma_fifo\",\"tiletype\":\"aie\",\"column\":{\"type\":\"evaluable\",\"expr\":\"30\",\"value\":30},\"row\":{\"type\":\"evaluable\",\"expr\":\"1\",\"value\":1},\"address\":{\"type\":\"evaluable\",\"expr\":\"0x0000\",\"value\":0},\"identifier\":\"0\",\"size\":{\"type\":\"evaluable\",\"expr\":\"512\",\"value\":512}},\"equality\":true}]"  deprecateConstraints=0
  FIFO8_2 : aieBasic/FIFO  FifoDepth=512  FIFOType=0  TileType=0  RowLocation=0  ColLocation=0  channel=0  blockJsonConstraints="[{\"type\":\"constraint\",\"constraintType\":\"location_fifo\",\"sid\":\"1278\",\"lhs\":{\"type\":\"location\",\"templParam\":\"fifo\",\"args\":{\"type\":\"fifo\",\"name\":\"DualStreamSSR/SSR8/FIFO8_2\",\"sid\":\"1278\"}},\"rhs\":{\"type\":\"fifogroup\",\"fifotype\":\"dma_fifo\",\"tiletype\":\"aie\",\"column\":{\"type\":\"evaluable\",\"expr\":\"30\",\"value\":30},\"row\":{\"type\":\"evaluable\",\"expr\":\"1\",\"value\":1},\"address\":{\"type\":\"evaluable\",\"expr\":\"0x2000\",\"value\":8192},\"identifier\":\"0\",\"size\":{\"type\":\"evaluable\",\"expr\":\"512\",\"value\":512}},\"equality\":true}]"  deprecateConstraints=0
  FIFO9_1 : aieBasic/FIFO  FifoDepth=512  FIFOType=0  TileType=0  RowLocation=0  ColLocation=0  channel=0  blockJsonConstraints="[{\"type\":\"constraint\",\"constraintType\":\"location_fifo\",\"sid\":\"1195\",\"lhs\":{\"type\":\"location\",\"templParam\":\"fifo\",\"args\":{\"type\":\"fifo\",\"name\":\"DualStreamSSR/SSR8/FIFO9_1\",\"sid\":\"1195\"}},\"rhs\":{\"type\":\"fifogroup\",\"fifotype\":\"dma_fifo\",\"tiletype\":\"aie\",\"column\":{\"type\":\"evaluable\",\"expr\":\"25\",\"value\":25},\"row\":{\"type\":\"evaluable\",\"expr\":\"1\",\"value\":1},\"address\":{\"type\":\"evaluable\",\"expr\":\"0x0000\",\"value\":0},\"identifier\":\"0\",\"size\":{\"type\":\"evaluable\",\"expr\":\"512\",\"value\":512}},\"equality\":true}]"  deprecateConstraints=0
  FIFO9_2 : aieBasic/FIFO  FifoDepth=512  FIFOType=0  TileType=0  RowLocation=0  ColLocation=0  channel=0  blockJsonConstraints="[{\"type\":\"constraint\",\"constraintType\":\"location_fifo\",\"sid\":\"1197\",\"lhs\":{\"type\":\"location\",\"templParam\":\"fifo\",\"args\":{\"type\":\"fifo\",\"name\":\"DualStreamSSR/SSR8/FIFO9_2\",\"sid\":\"1197\"}},\"rhs\":{\"type\":\"fifogroup\",\"fifotype\":\"dma_fifo\",\"tiletype\":\"aie\",\"column\":{\"type\":\"evaluable\",\"expr\":\"25\",\"value\":25},\"row\":{\"type\":\"evaluable\",\"expr\":\"1\",\"value\":1},\"address\":{\"type\":\"evaluable\",\"expr\":\"0x2000\",\"value\":8192},\"identifier\":\"0\",\"size\":{\"type\":\"evaluable\",\"expr\":\"512\",\"value\":512}},\"equality\":true}]"  deprecateConstraints=0
  PLIO{,1..9,12..13,16..17,20..21,24..25,28..29,32..33,36..37,40..47} (32 alike) : aieBasic/PLIO  PlioWidth=64  PlioFreqSpec=off  PlioFreq=250  ColLocation=0  channel=0  blockJsonConstraints=[]  deprecateConstraints=0
  filter : aieBasic/AIE Class Kernel  KernelAllAttrs=|  PortNames={'sin1'; 'sin2'; 'cout'}  PortSerializedTypes={'{Q2{P{Tinput_stream{1{t{Scint16}}}}}}'; '{Q2{P{Tinput_stream{1{t{Scint16}}}}}}'; '{P{Toutput_stream{1{t{Scacc48_t}}}}}'}  PortWindowSizes={0.000000000000000000e+00; 0.000000000000000000e+00; 0.000000000000000000e+00}  PortWindowMargins={0.000000000000000000e+00; 0.000000000000000000e+00; 0.000000000000000000e+00}  PortSynchronicities={'auto', 'auto', 'auto'}  PortSignalSizes={0.000000000000000000e+00; 0.000000000000000000e+00; 8.000000000000000000e+00}  ClassTemplateSpecKind=implicit  ClassTemplateParamNames={'NSamples'; 'ShiftAcc'; 'DiscardSample'; 'SwapRead'}  ClassTemplateParamKinds={'nontype'; 'nontype'; 'nontype'; 'nontype'}  ClassTemplateParamTypes={'int'; 'int'; 'bool'; 'bool'}  ClassTemplateParamValues={'512', '15', '0', '0'}  ClassCtorParamNames={'taps'}  ClassCtorParamSerializedTypes={'{R{Q1{C{Scint16}4}}}'}  ClassCtorParamValues={'[-54-21i 102-525i 8773-2748i 342+439i]'}  ClassIndex=1  ClassCtorIndex=1  ClassTabVisible=on  ClassTemplateParamsVisible=on  ClassCtorDeclVisible=on  ClassCtorParamsVisible=on  FunctionTabVisible=on  FunctionDecl=|  PortAttrs={ 'input', 'sin1', 'input_stream_cint16 * restrict', '', '', '', ''; 'input', 'sin2', 'input_stream_cint16 * restrict', '', '', '', ''; 'output', 'cout', 'output_stream< cacc48_t > *', '', '', '', 'OUTPUT_SIZE' }  PortAttrsEnables={'off', 'off', 'off', 'off', 'off', 'off', 'off';'off', 'off', 'off', 'off', 'off', 'off', 'off';'off', 'off', 'off', 'off', 'off', 'off', 'on'}  SampleTime=-1  ClassDeclTypeOptions=|  ClassDecl=|  ClassTemplateParams={ 'NSamples', 'int', 'BURST_LENGTH'; 'ShiftAcc', 'int', 'SHIFT_ACC'; 'DiscardSample', 'bool', 'FALSE'; 'SwapRead', 'bool', 'FALSE' }  ClassTemplateParamsEnables={'off', 'off', 'on';'off', 'off', 'on';'off', 'off', 'on';'off', 'off', 'on'}  ClassCtorDeclTypeOptions=C[1 1]@t51@FIR_MultiKernel_cout(cint16 const ( & taps ) [ 4 ])  ClassCtorDecl=FIR_MultiKernel_cout(cint16 const ( & taps ) [ 4 ])  ClassCtorParams={ 'taps', 'cint16 const ( &) [ 4 ]', 'phi_0' }  KernelHeaderFile=FirDoubleStream.h  KernelClassName=DoubleStream::FIR_MultiKernel_cout  KernelFunction=filter  KernelSourceFile=FirDoubleStream.cpp  KernelSearchPaths={'$SRC/aie_kernels'}  PreProcOptions={}  blockJsonConstraints="{\"type\":\"constraint\",\"constraintType\":\"location_kernel\",\"sid\":\"789\",\"lhs\":{\"type\":\"location\",\"templParam\":\"kernel\",\"args\":{\"type\":\"kernel\",\"name\":\"DualStreamSSR/SSR8/filter\",\"sid\":\"789\"}},\"rhs\":{\"type\":\"tile\",\"args\":[{\"type\":\"evaluable\",\"expr\":\"23\",\"value\":23},{\"type\":\"evaluable\",\"expr\":\"0\",\"value\":0}]},\"equality\":true}"
      KernelAllAttrs=|
      | s[12;12;9;9;19;14;21;23;24;21;12;24;26;26;26;27;28;9;21;23;23;23;24;25;14;19;19;29]@FunctionNameDeclFileNamePortNamesPortTypesPortSerializedTypesPortDirectionsPortWindowSizeEnablesPortWindowMarginEnablesPortSynchronicityEnablesPortSignalSizeEnablesFunctionDeclFunctionTemplateSpecKindFunctionTemplateParamNamesFunctionTemplateParamKindsFunctionTemplateParamTypesFunctionTemplateParamValuesFunctionTemplateParamEnablesClassDeclClassTemplateSpecKindClassTemplateParamNamesClassTemplateParamKindsClassTemplateParamTypesClassTemplateParamValuesClassTemplateParamEnablesClassCtorDeclsClassCtorParamNamesClassCtorParamTypesClassCtorParamSerializedTypes[1 1]@C[28 1]@t6@filtert42@../../../aie/aie_kernels/FirDoubleStream.hC[3 1]@t4@sin1t4@sin2t4@coutC[3 1]@t30@input_stream_cint16 * restrictt30@input_stream_cint16 * restrictt27@output_stream< cacc48_t > *C[3 1]@t37@{Q2{P{Tinput_stream{1{t{Scint16}}}}}}t37@{Q2{P{Tinput_stream{1{t{Scint16}}}}}}t36@{P{Toutput_stream{1{t{Scacc48_t}}}}}C[3 1]@t5@inputt5@inputt6@outputC[3 1]@l0@l0@l0@C[3 1]@l0@l0@l0@C[3 1]@l0@l0@l0@C[3 1]@l0@l0@l1@t246@namespace DoubleStream {
      | template < int NSamples, int ShiftAcc, bool DiscardSample, bool SwapRead > 
      | void FIR_MultiKernel_cout::
      | filter(input_stream_cint16 * restrict sin1, input_stream_cint16 * restrict sin2, output_stream< cacc48_t > * cout);
      | }t4@nonee[0 1]@e[0 1]@e[0 1]@e[0 1]@e[0 1]@t129@namespace DoubleStream {
      | template < int NSamples, int ShiftAcc, bool DiscardSample, bool SwapRead > class FIR_MultiKernel_cout;
      | }t8@implicitC[4 1]@t8@NSamplest8@ShiftAcct13@DiscardSamplet8@SwapReadC[4 1]@t7@nontypet7@nontypet7@nontypet7@nontypeC[4 1]@t3@intt3@intt4@boolt4@boolC[4 1]@nnnnC[4 1]@l1@l1@l1@l1@C[1 1]@t51@FIR_MultiKernel_cout(cint16 const ( & taps ) [ 4 ])C[1 1]@C[1 1]@t4@tapsC[1 1]@C[1 1]@t23@cint16 const ( &) [ 4 ]C[1 1]@C[1 1]@t20@{R{Q1{C{Scint16}4}}}
      FunctionDecl=|
      | namespace DoubleStream {
      | template < int NSamples, int ShiftAcc, bool DiscardSample, bool SwapRead > 
      | void FIR_MultiKernel_cout::
      | filter(input_stream_cint16 * restrict sin1, input_stream_cint16 * restrict sin2, output_stream< cacc48_t > * cout);
      | }
      ClassDeclTypeOptions=|
      | C[1 1]@t129@namespace DoubleStream {
      | template < int NSamples, int ShiftAcc, bool DiscardSample, bool SwapRead > class FIR_MultiKernel_cout;
      | }
      ClassDecl=|
      | namespace DoubleStream {
      | template < int NSamples, int ShiftAcc, bool DiscardSample, bool SwapRead > class FIR_MultiKernel_cout;
      | }
  filter1 : aieBasic/AIE Class Kernel  KernelAllAttrs=|  PortNames={'sin1'; 'sin2'; 'cin'; 'cout'}  PortSerializedTypes={'{Q2{P{Tinput_stream{1{t{Scint16}}}}}}'; '{Q2{P{Tinput_stream{1{t{Scint16}}}}}}'; '{P{Tinput_stream{1{t{Scacc48_t}}}}}'; '{P{Toutput_stream{1{t{Scacc48_t}}}}}'}  PortWindowSizes={0.000000000000000000e+00; 0.000000000000000000e+00; 0.000000000000000000e+00; 0.000000000000000000e+00}  PortWindowMargins={0.000000000000000000e+00; 0.000000000000000000e+00; 0.000000000000000000e+00; 0.000000000000000000e+00}  PortSynchronicities={'auto', 'auto', 'auto', 'auto'}  PortSignalSizes={0.000000000000000000e+00; 0.000000000000000000e+00; 0.000000000000000000e+00; 8.000000000000000000e+00}  ClassTemplateSpecKind=implicit  ClassTemplateParamNames={'NSamples'; 'ShiftAcc'; 'DiscardSample'; 'SwapRead'}  ClassTemplateParamKinds={'nontype'; 'nontype'; 'nontype'; 'nontype'}  ClassTemplateParamTypes={'int'; 'int'; 'bool'; 'bool'}  ClassTemplateParamValues={'512', '15', '0', '0'}  ClassCtorParamNames={'taps'}  ClassCtorParamSerializedTypes={'{R{Q1{C{Scint16}4}}}'}  ClassCtorParamValues={'[-83+21i 237+54i 4086-5221i 146+91i]'}  ClassIndex=1  ClassCtorIndex=1  ClassTabVisible=on  ClassTemplateParamsVisible=on  ClassCtorDeclVisible=on  ClassCtorParamsVisible=on  FunctionTabVisible=on  FunctionDecl=|  PortAttrs={ 'input', 'sin1', 'input_stream_cint16 * restrict', '', '', '', ''; 'input', 'sin2', 'input_stream_cint16 * restrict', '', '', '', ''; 'input', 'cin', 'input_stream< cacc48_t > *', '', '', '', ''; 'output', 'cout', 'output_stream< cacc48_t > *', '', '', '', 'OUTPUT_SIZE' }  PortAttrsEnables={'off', 'off', 'off', 'off', 'off', 'off', 'off';'off', 'off', 'off', 'off', 'off', 'off', 'off';'off', 'off', 'off', 'off', 'off', 'off', 'off';'off', 'off', 'off', 'off', 'off', 'off', 'on'}  SampleTime=-1  ClassDeclTypeOptions=|  ClassDecl=|  ClassTemplateParams={ 'NSamples', 'int', 'BURST_LENGTH'; 'ShiftAcc', 'int', 'SHIFT_ACC'; 'DiscardSample', 'bool', 'FALSE'; 'SwapRead', 'bool', 'FALSE' }  ClassTemplateParamsEnables={'off', 'off', 'on';'off', 'off', 'on';'off', 'off', 'on';'off', 'off', 'on'}  ClassCtorDeclTypeOptions=C[1 1]@t54@FIR_MultiKernel_cincout(cint16 const ( & taps ) [ 4 ])  ClassCtorDecl=FIR_MultiKernel_cincout(cint16 const ( & taps ) [ 4 ])  ClassCtorParams={ 'taps', 'cint16 const ( &) [ 4 ]', 'phi_1' }  KernelHeaderFile=FirDoubleStream.h  KernelClassName=DoubleStream::FIR_MultiKernel_cincout  KernelFunction=filter  KernelSourceFile=FirDoubleStream.cpp  KernelSearchPaths={'$SRC/aie_kernels'}  PreProcOptions={}  blockJsonConstraints="{\"type\":\"constraint\",\"constraintType\":\"location_kernel\",\"sid\":\"790\",\"lhs\":{\"type\":\"location\",\"templParam\":\"kernel\",\"args\":{\"type\":\"kernel\",\"name\":\"DualStreamSSR/SSR8/filter1\",\"sid\":\"790\"}},\"rhs\":{\"type\":\"tile\",\"args\":[{\"type\":\"evaluable\",\"expr\":\"24\",\"value\":24},{\"type\":\"evaluable\",\"expr\":\"0\",\"value\":0}]},\"equality\":true}"
      KernelAllAttrs=|
      | s[12;12;9;9;19;14;21;23;24;21;12;24;26;26;26;27;28;9;21;23;23;23;24;25;14;19;19;29]@FunctionNameDeclFileNamePortNamesPortTypesPortSerializedTypesPortDirectionsPortWindowSizeEnablesPortWindowMarginEnablesPortSynchronicityEnablesPortSignalSizeEnablesFunctionDeclFunctionTemplateSpecKindFunctionTemplateParamNamesFunctionTemplateParamKindsFunctionTemplateParamTypesFunctionTemplateParamValuesFunctionTemplateParamEnablesClassDeclClassTemplateSpecKindClassTemplateParamNamesClassTemplateParamKindsClassTemplateParamTypesClassTemplateParamValuesClassTemplateParamEnablesClassCtorDeclsClassCtorParamNamesClassCtorParamTypesClassCtorParamSerializedTypes[1 1]@C[28 1]@t6@filtert42@../../../aie/aie_kernels/FirDoubleStream.hC[4 1]@t4@sin1t4@sin2t3@cint4@coutC[4 1]@t30@input_stream_cint16 * restrictt30@input_stream_cint16 * restrictt26@input_stream< cacc48_t > *t27@output_stream< cacc48_t > *C[4 1]@t37@{Q2{P{Tinput_stream{1{t{Scint16}}}}}}t37@{Q2{P{Tinput_stream{1{t{Scint16}}}}}}t35@{P{Tinput_stream{1{t{Scacc48_t}}}}}t36@{P{Toutput_stream{1{t{Scacc48_t}}}}}C[4 1]@t5@inputt5@inputt5@inputt6@outputC[4 1]@l0@l0@l0@l0@C[4 1]@l0@l0@l0@l0@C[4 1]@l0@l0@l0@l0@C[4 1]@l0@l0@l0@l1@t281@namespace DoubleStream {
      | template < int NSamples, int ShiftAcc, bool DiscardSample, bool SwapRead > 
      | void FIR_MultiKernel_cincout::
      | filter(input_stream_cint16 * restrict sin1, input_stream_cint16 * restrict sin2, input_stream< cacc48_t > * cin, output_stream< cacc48_t > * cout);
      | }t4@nonee[0 1]@e[0 1]@e[0 1]@e[0 1]@e[0 1]@t132@namespace DoubleStream {
      | template < int NSamples, int ShiftAcc, bool DiscardSample, bool SwapRead > class FIR_MultiKernel_cincout;
      | }t8@implicitC[4 1]@t8@NSamplest8@ShiftAcct13@DiscardSamplet8@SwapReadC[4 1]@t7@nontypet7@nontypet7@nontypet7@nontypeC[4 1]@t3@intt3@intt4@boolt4@boolC[4 1]@nnnnC[4 1]@l1@l1@l1@l1@C[1 1]@t54@FIR_MultiKernel_cincout(cint16 const ( & taps ) [ 4 ])C[1 1]@C[1 1]@t4@tapsC[1 1]@C[1 1]@t23@cint16 const ( &) [ 4 ]C[1 1]@C[1 1]@t20@{R{Q1{C{Scint16}4}}}
      FunctionDecl=|
      | namespace DoubleStream {
      | template < int NSamples, int ShiftAcc, bool DiscardSample, bool SwapRead > 
      | void FIR_MultiKernel_cincout::
      | filter(input_stream_cint16 * restrict sin1, input_stream_cint16 * restrict sin2, input_stream< cacc48_t > * cin, output_stream< cacc48_t > * cout);
      | }
      ClassDeclTypeOptions=|
      | C[1 1]@t132@namespace DoubleStream {
      | template < int NSamples, int ShiftAcc, bool DiscardSample, bool SwapRead > class FIR_MultiKernel_cincout;
      | }
      ClassDecl=|
      | namespace DoubleStream {
      | template < int NSamples, int ShiftAcc, bool DiscardSample, bool SwapRead > class FIR_MultiKernel_cincout;
      | }
  filter10 : aieBasic/AIE Class Kernel  KernelAllAttrs=|  PortNames={'sin1'; 'sin2'; 'cin'; 'cout'}  PortSerializedTypes={'{Q2{P{Tinput_stream{1{t{Scint16}}}}}}'; '{Q2{P{Tinput_stream{1{t{Scint16}}}}}}'; '{P{Tinput_stream{1{t{Scacc48_t}}}}}'; '{P{Toutput_stream{1{t{Scacc48_t}}}}}'}  PortWindowSizes={0.000000000000000000e+00; 0.000000000000000000e+00; 0.000000000000000000e+00; 0.000000000000000000e+00}  PortWindowMargins={0.000000000000000000e+00; 0.000000000000000000e+00; 0.000000000000000000e+00; 0.000000000000000000e+00}  PortSynchronicities={'auto', 'auto', 'auto', 'auto'}  PortSignalSizes={0.000000000000000000e+00; 0.000000000000000000e+00; 0.000000000000000000e+00; 8.000000000000000000e+00}  ClassTemplateSpecKind=implicit  ClassTemplateParamNames={'NSamples'; 'ShiftAcc'; 'DiscardSample'; 'SwapRead'}  ClassTemplateParamKinds={'nontype'; 'nontype'; 'nontype'; 'nontype'}  ClassTemplateParamTypes={'int'; 'int'; 'bool'; 'bool'}  ClassTemplateParamValues={'512', '15', '0', '0'}  ClassCtorParamNames={'taps'}  ClassCtorParamSerializedTypes={'{R{Q1{C{Scint16}4}}}'}  ClassCtorParamValues={'[-21+26i 1183+239i 248-2878i -160+111i]'}  ClassIndex=1  ClassCtorIndex=1  ClassTabVisible=on  ClassTemplateParamsVisible=on  ClassCtorDeclVisible=on  ClassCtorParamsVisible=on  FunctionTabVisible=on  FunctionDecl=|  PortAttrs={ 'input', 'sin1', 'input_stream_cint16 * restrict', '', '', '', ''; 'input', 'sin2', 'input_stream_cint16 * restrict', '', '', '', ''; 'input', 'cin', 'input_stream< cacc48_t > *', '', '', '', ''; 'output', 'cout', 'output_stream< cacc48_t > *', '', '', '', 'OUTPUT_SIZE' }  PortAttrsEnables={'off', 'off', 'off', 'off', 'off', 'off', 'off';'off', 'off', 'off', 'off', 'off', 'off', 'off';'off', 'off', 'off', 'off', 'off', 'off', 'off';'off', 'off', 'off', 'off', 'off', 'off', 'on'}  SampleTime=-1  ClassDeclTypeOptions=|  ClassDecl=|  ClassTemplateParams={ 'NSamples', 'int', 'BURST_LENGTH'; 'ShiftAcc', 'int', 'SHIFT_ACC'; 'DiscardSample', 'bool', 'FALSE'; 'SwapRead', 'bool', 'FALSE' }  ClassTemplateParamsEnables={'off', 'off', 'on';'off', 'off', 'on';'off', 'off', 'on';'off', 'off', 'on'}  ClassCtorDeclTypeOptions=C[1 1]@t54@FIR_MultiKernel_cincout(cint16 const ( & taps ) [ 4 ])  ClassCtorDecl=FIR_MultiKernel_cincout(cint16 const ( & taps ) [ 4 ])  ClassCtorParams={ 'taps', 'cint16 const ( &) [ 4 ]', 'phi_2' }  KernelHeaderFile=FirDoubleStream.h  KernelClassName=DoubleStream::FIR_MultiKernel_cincout  KernelFunction=filter  KernelSourceFile=FirDoubleStream.cpp  KernelSearchPaths={'$SRC/aie_kernels'}  PreProcOptions={}  blockJsonConstraints="{\"type\":\"constraint\",\"constraintType\":\"location_kernel\",\"sid\":\"791\",\"lhs\":{\"type\":\"location\",\"templParam\":\"kernel\",\"args\":{\"type\":\"kernel\",\"name\":\"DualStreamSSR/SSR8/filter10\",\"sid\":\"791\"}},\"rhs\":{\"type\":\"tile\",\"args\":[{\"type\":\"evaluable\",\"expr\":\"26\",\"value\":26},{\"type\":\"evaluable\",\"expr\":\"1\",\"value\":1}]},\"equality\":true}"
      KernelAllAttrs=|
      | s[12;12;9;9;19;14;21;23;24;21;12;24;26;26;26;27;28;9;21;23;23;23;24;25;14;19;19;29]@FunctionNameDeclFileNamePortNamesPortTypesPortSerializedTypesPortDirectionsPortWindowSizeEnablesPortWindowMarginEnablesPortSynchronicityEnablesPortSignalSizeEnablesFunctionDeclFunctionTemplateSpecKindFunctionTemplateParamNamesFunctionTemplateParamKindsFunctionTemplateParamTypesFunctionTemplateParamValuesFunctionTemplateParamEnablesClassDeclClassTemplateSpecKindClassTemplateParamNamesClassTemplateParamKindsClassTemplateParamTypesClassTemplateParamValuesClassTemplateParamEnablesClassCtorDeclsClassCtorParamNamesClassCtorParamTypesClassCtorParamSerializedTypes[1 1]@C[28 1]@t6@filtert42@../../../aie/aie_kernels/FirDoubleStream.hC[4 1]@t4@sin1t4@sin2t3@cint4@coutC[4 1]@t30@input_stream_cint16 * restrictt30@input_stream_cint16 * restrictt26@input_stream< cacc48_t > *t27@output_stream< cacc48_t > *C[4 1]@t37@{Q2{P{Tinput_stream{1{t{Scint16}}}}}}t37@{Q2{P{Tinput_stream{1{t{Scint16}}}}}}t35@{P{Tinput_stream{1{t{Scacc48_t}}}}}t36@{P{Toutput_stream{1{t{Scacc48_t}}}}}C[4 1]@t5@inputt5@inputt5@inputt6@outputC[4 1]@l0@l0@l0@l0@C[4 1]@l0@l0@l0@l0@C[4 1]@l0@l0@l0@l0@C[4 1]@l0@l0@l0@l1@t281@namespace DoubleStream {
      | template < int NSamples, int ShiftAcc, bool DiscardSample, bool SwapRead > 
      | void FIR_MultiKernel_cincout::
      | filter(input_stream_cint16 * restrict sin1, input_stream_cint16 * restrict sin2, input_stream< cacc48_t > * cin, output_stream< cacc48_t > * cout);
      | }t4@nonee[0 1]@e[0 1]@e[0 1]@e[0 1]@e[0 1]@t132@namespace DoubleStream {
      | template < int NSamples, int ShiftAcc, bool DiscardSample, bool SwapRead > class FIR_MultiKernel_cincout;
      | }t8@implicitC[4 1]@t8@NSamplest8@ShiftAcct13@DiscardSamplet8@SwapReadC[4 1]@t7@nontypet7@nontypet7@nontypet7@nontypeC[4 1]@t3@intt3@intt4@boolt4@boolC[4 1]@nnnnC[4 1]@l1@l1@l1@l1@C[1 1]@t54@FIR_MultiKernel_cincout(cint16 const ( & taps ) [ 4 ])C[1 1]@C[1 1]@t4@tapsC[1 1]@C[1 1]@t23@cint16 const ( &) [ 4 ]C[1 1]@C[1 1]@t20@{R{Q1{C{Scint16}4}}}
      FunctionDecl=|
      | namespace DoubleStream {
      | template < int NSamples, int ShiftAcc, bool DiscardSample, bool SwapRead > 
      | void FIR_MultiKernel_cincout::
      | filter(input_stream_cint16 * restrict sin1, input_stream_cint16 * restrict sin2, input_stream< cacc48_t > * cin, output_stream< cacc48_t > * cout);
      | }
      ClassDeclTypeOptions=|
      | C[1 1]@t132@namespace DoubleStream {
      | template < int NSamples, int ShiftAcc, bool DiscardSample, bool SwapRead > class FIR_MultiKernel_cincout;
      | }
      ClassDecl=|
      | namespace DoubleStream {
      | template < int NSamples, int ShiftAcc, bool DiscardSample, bool SwapRead > class FIR_MultiKernel_cincout;
      | }
  filter11 : aieBasic/AIE Class Kernel  KernelAllAttrs=|  PortNames={'sin1'; 'sin2'; 'cin'; 'cout'}  PortSerializedTypes={'{Q2{P{Tinput_stream{1{t{Scint16}}}}}}'; '{Q2{P{Tinput_stream{1{t{Scint16}}}}}}'; '{P{Tinput_stream{1{t{Scacc48_t}}}}}'; '{P{Toutput_stream{1{t{Scacc48_t}}}}}'}  PortWindowSizes={0.000000000000000000e+00; 0.000000000000000000e+00; 0.000000000000000000e+00; 0.000000000000000000e+00}  PortWindowMargins={0.000000000000000000e+00; 0.000000000000000000e+00; 0.000000000000000000e+00; 0.000000000000000000e+00}  PortSynchronicities={'auto', 'auto', 'auto', 'auto'}  PortSignalSizes={0.000000000000000000e+00; 0.000000000000000000e+00; 0.000000000000000000e+00; 8.000000000000000000e+00}  ClassTemplateSpecKind=implicit  ClassTemplateParamNames={'NSamples'; 'ShiftAcc'; 'DiscardSample'; 'SwapRead'}  ClassTemplateParamKinds={'nontype'; 'nontype'; 'nontype'; 'nontype'}  ClassTemplateParamTypes={'int'; 'int'; 'bool'; 'bool'}  ClassTemplateParamValues={'512', '15', '0', '0'}  ClassCtorParamNames={'taps'}  ClassCtorParamSerializedTypes={'{R{Q1{C{Scint16}4}}}'}  ClassCtorParamValues={'[14-121i 1454-497i 237+96i -121+233i]'}  ClassIndex=1  ClassCtorIndex=1  ClassTabVisible=on  ClassTemplateParamsVisible=on  ClassCtorDeclVisible=on  ClassCtorParamsVisible=on  FunctionTabVisible=on  FunctionDecl=|  PortAttrs={ 'input', 'sin1', 'input_stream_cint16 * restrict', '', '', '', ''; 'input', 'sin2', 'input_stream_cint16 * restrict', '', '', '', ''; 'input', 'cin', 'input_stream< cacc48_t > *', '', '', '', ''; 'output', 'cout', 'output_stream< cacc48_t > *', '', '', '', 'OUTPUT_SIZE' }  PortAttrsEnables={'off', 'off', 'off', 'off', 'off', 'off', 'off';'off', 'off', 'off', 'off', 'off', 'off', 'off';'off', 'off', 'off', 'off', 'off', 'off', 'off';'off', 'off', 'off', 'off', 'off', 'off', 'on'}  SampleTime=-1  ClassDeclTypeOptions=|  ClassDecl=|  ClassTemplateParams={ 'NSamples', 'int', 'BURST_LENGTH'; 'ShiftAcc', 'int', 'SHIFT_ACC'; 'DiscardSample', 'bool', 'FALSE'; 'SwapRead', 'bool', 'FALSE' }  ClassTemplateParamsEnables={'off', 'off', 'on';'off', 'off', 'on';'off', 'off', 'on';'off', 'off', 'on'}  ClassCtorDeclTypeOptions=C[1 1]@t54@FIR_MultiKernel_cincout(cint16 const ( & taps ) [ 4 ])  ClassCtorDecl=FIR_MultiKernel_cincout(cint16 const ( & taps ) [ 4 ])  ClassCtorParams={ 'taps', 'cint16 const ( &) [ 4 ]', 'phi_3' }  KernelHeaderFile=FirDoubleStream.h  KernelClassName=DoubleStream::FIR_MultiKernel_cincout  KernelFunction=filter  KernelSourceFile=FirDoubleStream.cpp  KernelSearchPaths={'$SRC/aie_kernels'}  PreProcOptions={}  blockJsonConstraints="{\"type\":\"constraint\",\"constraintType\":\"location_kernel\",\"sid\":\"792\",\"lhs\":{\"type\":\"location\",\"templParam\":\"kernel\",\"args\":{\"type\":\"kernel\",\"name\":\"DualStreamSSR/SSR8/filter11\",\"sid\":\"792\"}},\"rhs\":{\"type\":\"tile\",\"args\":[{\"type\":\"evaluable\",\"expr\":\"27\",\"value\":27},{\"type\":\"evaluable\",\"expr\":\"1\",\"value\":1}]},\"equality\":true}"
      KernelAllAttrs=|
      | s[12;12;9;9;19;14;21;23;24;21;12;24;26;26;26;27;28;9;21;23;23;23;24;25;14;19;19;29]@FunctionNameDeclFileNamePortNamesPortTypesPortSerializedTypesPortDirectionsPortWindowSizeEnablesPortWindowMarginEnablesPortSynchronicityEnablesPortSignalSizeEnablesFunctionDeclFunctionTemplateSpecKindFunctionTemplateParamNamesFunctionTemplateParamKindsFunctionTemplateParamTypesFunctionTemplateParamValuesFunctionTemplateParamEnablesClassDeclClassTemplateSpecKindClassTemplateParamNamesClassTemplateParamKindsClassTemplateParamTypesClassTemplateParamValuesClassTemplateParamEnablesClassCtorDeclsClassCtorParamNamesClassCtorParamTypesClassCtorParamSerializedTypes[1 1]@C[28 1]@t6@filtert42@../../../aie/aie_kernels/FirDoubleStream.hC[4 1]@t4@sin1t4@sin2t3@cint4@coutC[4 1]@t30@input_stream_cint16 * restrictt30@input_stream_cint16 * restrictt26@input_stream< cacc48_t > *t27@output_stream< cacc48_t > *C[4 1]@t37@{Q2{P{Tinput_stream{1{t{Scint16}}}}}}t37@{Q2{P{Tinput_stream{1{t{Scint16}}}}}}t35@{P{Tinput_stream{1{t{Scacc48_t}}}}}t36@{P{Toutput_stream{1{t{Scacc48_t}}}}}C[4 1]@t5@inputt5@inputt5@inputt6@outputC[4 1]@l0@l0@l0@l0@C[4 1]@l0@l0@l0@l0@C[4 1]@l0@l0@l0@l0@C[4 1]@l0@l0@l0@l1@t281@namespace DoubleStream {
      | template < int NSamples, int ShiftAcc, bool DiscardSample, bool SwapRead > 
      | void FIR_MultiKernel_cincout::
      | filter(input_stream_cint16 * restrict sin1, input_stream_cint16 * restrict sin2, input_stream< cacc48_t > * cin, output_stream< cacc48_t > * cout);
      | }t4@nonee[0 1]@e[0 1]@e[0 1]@e[0 1]@e[0 1]@t132@namespace DoubleStream {
      | template < int NSamples, int ShiftAcc, bool DiscardSample, bool SwapRead > class FIR_MultiKernel_cincout;
      | }t8@implicitC[4 1]@t8@NSamplest8@ShiftAcct13@DiscardSamplet8@SwapReadC[4 1]@t7@nontypet7@nontypet7@nontypet7@nontypeC[4 1]@t3@intt3@intt4@boolt4@boolC[4 1]@nnnnC[4 1]@l1@l1@l1@l1@C[1 1]@t54@FIR_MultiKernel_cincout(cint16 const ( & taps ) [ 4 ])C[1 1]@C[1 1]@t4@tapsC[1 1]@C[1 1]@t23@cint16 const ( &) [ 4 ]C[1 1]@C[1 1]@t20@{R{Q1{C{Scint16}4}}}
      FunctionDecl=|
      | namespace DoubleStream {
      | template < int NSamples, int ShiftAcc, bool DiscardSample, bool SwapRead > 
      | void FIR_MultiKernel_cincout::
      | filter(input_stream_cint16 * restrict sin1, input_stream_cint16 * restrict sin2, input_stream< cacc48_t > * cin, output_stream< cacc48_t > * cout);
      | }
      ClassDeclTypeOptions=|
      | C[1 1]@t132@namespace DoubleStream {
      | template < int NSamples, int ShiftAcc, bool DiscardSample, bool SwapRead > class FIR_MultiKernel_cincout;
      | }
      ClassDecl=|
      | namespace DoubleStream {
      | template < int NSamples, int ShiftAcc, bool DiscardSample, bool SwapRead > class FIR_MultiKernel_cincout;
      | }
  filter12 : aieBasic/AIE Class Kernel  KernelAllAttrs=|  PortNames={'sin1'; 'sin2'; 'cin'; 'cout'}  PortSerializedTypes={'{Q2{P{Tinput_stream{1{t{Scint16}}}}}}'; '{Q2{P{Tinput_stream{1{t{Scint16}}}}}}'; '{P{Tinput_stream{1{t{Scacc48_t}}}}}'; '{P{Toutput_stream{1{t{Scacc48_t}}}}}'}  PortWindowSizes={0.000000000000000000e+00; 0.000000000000000000e+00; 0.000000000000000000e+00; 0.000000000000000000e+00}  PortWindowMargins={0.000000000000000000e+00; 0.000000000000000000e+00; 0.000000000000000000e+00; 0.000000000000000000e+00}  PortSynchronicities={'auto', 'auto', 'auto', 'auto'}  PortSignalSizes={0.000000000000000000e+00; 0.000000000000000000e+00; 0.000000000000000000e+00; 8.000000000000000000e+00}  ClassTemplateSpecKind=implicit  ClassTemplateParamNames={'NSamples'; 'ShiftAcc'; 'DiscardSample'; 'SwapRead'}  ClassTemplateParamKinds={'nontype'; 'nontype'; 'nontype'; 'nontype'}  ClassTemplateParamTypes={'int'; 'int'; 'bool'; 'bool'}  ClassTemplateParamValues={'512', '15', '0', '0'}  ClassCtorParamNames={'taps'}  ClassCtorParamSerializedTypes={'{R{Q1{C{Scint16}4}}}'}  ClassCtorParamValues={'[-121-233i 237-96i 1454+497i 14+121i]'}  ClassIndex=1  ClassCtorIndex=1  ClassTabVisible=on  ClassTemplateParamsVisible=on  ClassCtorDeclVisible=on  ClassCtorParamsVisible=on  FunctionTabVisible=on  FunctionDecl=|  PortAttrs={ 'input', 'sin1', 'input_stream_cint16 * restrict', '', '', '', ''; 'input', 'sin2', 'input_stream_cint16 * restrict', '', '', '', ''; 'input', 'cin', 'input_stream< cacc48_t > *', '', '', '', ''; 'output', 'cout', 'output_stream< cacc48_t > *', '', '', '', 'OUTPUT_SIZE' }  PortAttrsEnables={'off', 'off', 'off', 'off', 'off', 'off', 'off';'off', 'off', 'off', 'off', 'off', 'off', 'off';'off', 'off', 'off', 'off', 'off', 'off', 'off';'off', 'off', 'off', 'off', 'off', 'off', 'on'}  SampleTime=-1  ClassDeclTypeOptions=|  ClassDecl=|  ClassTemplateParams={ 'NSamples', 'int', 'BURST_LENGTH'; 'ShiftAcc', 'int', 'SHIFT_ACC'; 'DiscardSample', 'bool', 'FALSE'; 'SwapRead', 'bool', 'FALSE' }  ClassTemplateParamsEnables={'off', 'off', 'on';'off', 'off', 'on';'off', 'off', 'on';'off', 'off', 'on'}  ClassCtorDeclTypeOptions=C[1 1]@t54@FIR_MultiKernel_cincout(cint16 const ( & taps ) [ 4 ])  ClassCtorDecl=FIR_MultiKernel_cincout(cint16 const ( & taps ) [ 4 ])  ClassCtorParams={ 'taps', 'cint16 const ( &) [ 4 ]', 'phi_4' }  KernelHeaderFile=FirDoubleStream.h  KernelClassName=DoubleStream::FIR_MultiKernel_cincout  KernelFunction=filter  KernelSourceFile=FirDoubleStream.cpp  KernelSearchPaths={'$SRC/aie_kernels'}  PreProcOptions={}  blockJsonConstraints="{\"type\":\"constraint\",\"constraintType\":\"location_kernel\",\"sid\":\"793\",\"lhs\":{\"type\":\"location\",\"templParam\":\"kernel\",\"args\":{\"type\":\"kernel\",\"name\":\"DualStreamSSR/SSR8/filter12\",\"sid\":\"793\"}},\"rhs\":{\"type\":\"tile\",\"args\":[{\"type\":\"evaluable\",\"expr\":\"28\",\"value\":28},{\"type\":\"evaluable\",\"expr\":\"1\",\"value\":1}]},\"equality\":true}"
      KernelAllAttrs=|
      | s[12;12;9;9;19;14;21;23;24;21;12;24;26;26;26;27;28;9;21;23;23;23;24;25;14;19;19;29]@FunctionNameDeclFileNamePortNamesPortTypesPortSerializedTypesPortDirectionsPortWindowSizeEnablesPortWindowMarginEnablesPortSynchronicityEnablesPortSignalSizeEnablesFunctionDeclFunctionTemplateSpecKindFunctionTemplateParamNamesFunctionTemplateParamKindsFunctionTemplateParamTypesFunctionTemplateParamValuesFunctionTemplateParamEnablesClassDeclClassTemplateSpecKindClassTemplateParamNamesClassTemplateParamKindsClassTemplateParamTypesClassTemplateParamValuesClassTemplateParamEnablesClassCtorDeclsClassCtorParamNamesClassCtorParamTypesClassCtorParamSerializedTypes[1 1]@C[28 1]@t6@filtert42@../../../aie/aie_kernels/FirDoubleStream.hC[4 1]@t4@sin1t4@sin2t3@cint4@coutC[4 1]@t30@input_stream_cint16 * restrictt30@input_stream_cint16 * restrictt26@input_stream< cacc48_t > *t27@output_stream< cacc48_t > *C[4 1]@t37@{Q2{P{Tinput_stream{1{t{Scint16}}}}}}t37@{Q2{P{Tinput_stream{1{t{Scint16}}}}}}t35@{P{Tinput_stream{1{t{Scacc48_t}}}}}t36@{P{Toutput_stream{1{t{Scacc48_t}}}}}C[4 1]@t5@inputt5@inputt5@inputt6@outputC[4 1]@l0@l0@l0@l0@C[4 1]@l0@l0@l0@l0@C[4 1]@l0@l0@l0@l0@C[4 1]@l0@l0@l0@l1@t281@namespace DoubleStream {
      | template < int NSamples, int ShiftAcc, bool DiscardSample, bool SwapRead > 
      | void FIR_MultiKernel_cincout::
      | filter(input_stream_cint16 * restrict sin1, input_stream_cint16 * restrict sin2, input_stream< cacc48_t > * cin, output_stream< cacc48_t > * cout);
      | }t4@nonee[0 1]@e[0 1]@e[0 1]@e[0 1]@e[0 1]@t132@namespace DoubleStream {
      | template < int NSamples, int ShiftAcc, bool DiscardSample, bool SwapRead > class FIR_MultiKernel_cincout;
      | }t8@implicitC[4 1]@t8@NSamplest8@ShiftAcct13@DiscardSamplet8@SwapReadC[4 1]@t7@nontypet7@nontypet7@nontypet7@nontypeC[4 1]@t3@intt3@intt4@boolt4@boolC[4 1]@nnnnC[4 1]@l1@l1@l1@l1@C[1 1]@t54@FIR_MultiKernel_cincout(cint16 const ( & taps ) [ 4 ])C[1 1]@C[1 1]@t4@tapsC[1 1]@C[1 1]@t23@cint16 const ( &) [ 4 ]C[1 1]@C[1 1]@t20@{R{Q1{C{Scint16}4}}}
      FunctionDecl=|
      | namespace DoubleStream {
      | template < int NSamples, int ShiftAcc, bool DiscardSample, bool SwapRead > 
      | void FIR_MultiKernel_cincout::
      | filter(input_stream_cint16 * restrict sin1, input_stream_cint16 * restrict sin2, input_stream< cacc48_t > * cin, output_stream< cacc48_t > * cout);
      | }
      ClassDeclTypeOptions=|
      | C[1 1]@t132@namespace DoubleStream {
      | template < int NSamples, int ShiftAcc, bool DiscardSample, bool SwapRead > class FIR_MultiKernel_cincout;
      | }
      ClassDecl=|
      | namespace DoubleStream {
      | template < int NSamples, int ShiftAcc, bool DiscardSample, bool SwapRead > class FIR_MultiKernel_cincout;
      | }
  filter13 : aieBasic/AIE Class Kernel  KernelAllAttrs=|  PortNames={'sin1'; 'sin2'; 'cin'; 'cout'}  PortSerializedTypes={'{Q2{P{Tinput_stream{1{t{Scint16}}}}}}'; '{Q2{P{Tinput_stream{1{t{Scint16}}}}}}'; '{P{Tinput_stream{1{t{Scacc48_t}}}}}'; '{P{Toutput_stream{1{t{Scacc48_t}}}}}'}  PortWindowSizes={0.000000000000000000e+00; 0.000000000000000000e+00; 0.000000000000000000e+00; 0.000000000000000000e+00}  PortWindowMargins={0.000000000000000000e+00; 0.000000000000000000e+00; 0.000000000000000000e+00; 0.000000000000000000e+00}  PortSynchronicities={'auto', 'auto', 'auto', 'auto'}  PortSignalSizes={0.000000000000000000e+00; 0.000000000000000000e+00; 0.000000000000000000e+00; 8.000000000000000000e+00}  ClassTemplateSpecKind=implicit  ClassTemplateParamNames={'NSamples'; 'ShiftAcc'; 'DiscardSample'; 'SwapRead'}  ClassTemplateParamKinds={'nontype'; 'nontype'; 'nontype'; 'nontype'}  ClassTemplateParamTypes={'int'; 'int'; 'bool'; 'bool'}  ClassTemplateParamValues={'512', '15', '0', '0'}  ClassCtorParamNames={'taps'}  ClassCtorParamSerializedTypes={'{R{Q1{C{Scint16}4}}}'}  ClassCtorParamValues={'[-160-111i 248+2878i 1183-239i -21-26i]'}  ClassIndex=1  ClassCtorIndex=1  ClassTabVisible=on  ClassTemplateParamsVisible=on  ClassCtorDeclVisible=on  ClassCtorParamsVisible=on  FunctionTabVisible=on  FunctionDecl=|  PortAttrs={ 'input', 'sin1', 'input_stream_cint16 * restrict', '', '', '', ''; 'input', 'sin2', 'input_stream_cint16 * restrict', '', '', '', ''; 'input', 'cin', 'input_stream< cacc48_t > *', '', '', '', ''; 'output', 'cout', 'output_stream< cacc48_t > *', '', '', '', 'OUTPUT_SIZE' }  PortAttrsEnables={'off', 'off', 'off', 'off', 'off', 'off', 'off';'off', 'off', 'off', 'off', 'off', 'off', 'off';'off', 'off', 'off', 'off', 'off', 'off', 'off';'off', 'off', 'off', 'off', 'off', 'off', 'on'}  SampleTime=-1  ClassDeclTypeOptions=|  ClassDecl=|  ClassTemplateParams={ 'NSamples', 'int', 'BURST_LENGTH'; 'ShiftAcc', 'int', 'SHIFT_ACC'; 'DiscardSample', 'bool', 'FALSE'; 'SwapRead', 'bool', 'FALSE' }  ClassTemplateParamsEnables={'off', 'off', 'on';'off', 'off', 'on';'off', 'off', 'on';'off', 'off', 'on'}  ClassCtorDeclTypeOptions=C[1 1]@t54@FIR_MultiKernel_cincout(cint16 const ( & taps ) [ 4 ])  ClassCtorDecl=FIR_MultiKernel_cincout(cint16 const ( & taps ) [ 4 ])  ClassCtorParams={ 'taps', 'cint16 const ( &) [ 4 ]', 'phi_5' }  KernelHeaderFile=FirDoubleStream.h  KernelClassName=DoubleStream::FIR_MultiKernel_cincout  KernelFunction=filter  KernelSourceFile=FirDoubleStream.cpp  KernelSearchPaths={'$SRC/aie_kernels'}  PreProcOptions={}  blockJsonConstraints="{\"type\":\"constraint\",\"constraintType\":\"location_kernel\",\"sid\":\"794\",\"lhs\":{\"type\":\"location\",\"templParam\":\"kernel\",\"args\":{\"type\":\"kernel\",\"name\":\"DualStreamSSR/SSR8/filter13\",\"sid\":\"794\"}},\"rhs\":{\"type\":\"tile\",\"args\":[{\"type\":\"evaluable\",\"expr\":\"29\",\"value\":29},{\"type\":\"evaluable\",\"expr\":\"1\",\"value\":1}]},\"equality\":true}"
      KernelAllAttrs=|
      | s[12;12;9;9;19;14;21;23;24;21;12;24;26;26;26;27;28;9;21;23;23;23;24;25;14;19;19;29]@FunctionNameDeclFileNamePortNamesPortTypesPortSerializedTypesPortDirectionsPortWindowSizeEnablesPortWindowMarginEnablesPortSynchronicityEnablesPortSignalSizeEnablesFunctionDeclFunctionTemplateSpecKindFunctionTemplateParamNamesFunctionTemplateParamKindsFunctionTemplateParamTypesFunctionTemplateParamValuesFunctionTemplateParamEnablesClassDeclClassTemplateSpecKindClassTemplateParamNamesClassTemplateParamKindsClassTemplateParamTypesClassTemplateParamValuesClassTemplateParamEnablesClassCtorDeclsClassCtorParamNamesClassCtorParamTypesClassCtorParamSerializedTypes[1 1]@C[28 1]@t6@filtert42@../../../aie/aie_kernels/FirDoubleStream.hC[4 1]@t4@sin1t4@sin2t3@cint4@coutC[4 1]@t30@input_stream_cint16 * restrictt30@input_stream_cint16 * restrictt26@input_stream< cacc48_t > *t27@output_stream< cacc48_t > *C[4 1]@t37@{Q2{P{Tinput_stream{1{t{Scint16}}}}}}t37@{Q2{P{Tinput_stream{1{t{Scint16}}}}}}t35@{P{Tinput_stream{1{t{Scacc48_t}}}}}t36@{P{Toutput_stream{1{t{Scacc48_t}}}}}C[4 1]@t5@inputt5@inputt5@inputt6@outputC[4 1]@l0@l0@l0@l0@C[4 1]@l0@l0@l0@l0@C[4 1]@l0@l0@l0@l0@C[4 1]@l0@l0@l0@l1@t281@namespace DoubleStream {
      | template < int NSamples, int ShiftAcc, bool DiscardSample, bool SwapRead > 
      | void FIR_MultiKernel_cincout::
      | filter(input_stream_cint16 * restrict sin1, input_stream_cint16 * restrict sin2, input_stream< cacc48_t > * cin, output_stream< cacc48_t > * cout);
      | }t4@nonee[0 1]@e[0 1]@e[0 1]@e[0 1]@e[0 1]@t132@namespace DoubleStream {
      | template < int NSamples, int ShiftAcc, bool DiscardSample, bool SwapRead > class FIR_MultiKernel_cincout;
      | }t8@implicitC[4 1]@t8@NSamplest8@ShiftAcct13@DiscardSamplet8@SwapReadC[4 1]@t7@nontypet7@nontypet7@nontypet7@nontypeC[4 1]@t3@intt3@intt4@boolt4@boolC[4 1]@nnnnC[4 1]@l1@l1@l1@l1@C[1 1]@t54@FIR_MultiKernel_cincout(cint16 const ( & taps ) [ 4 ])C[1 1]@C[1 1]@t4@tapsC[1 1]@C[1 1]@t23@cint16 const ( &) [ 4 ]C[1 1]@C[1 1]@t20@{R{Q1{C{Scint16}4}}}
      FunctionDecl=|
      | namespace DoubleStream {
      | template < int NSamples, int ShiftAcc, bool DiscardSample, bool SwapRead > 
      | void FIR_MultiKernel_cincout::
      | filter(input_stream_cint16 * restrict sin1, input_stream_cint16 * restrict sin2, input_stream< cacc48_t > * cin, output_stream< cacc48_t > * cout);
      | }
      ClassDeclTypeOptions=|
      | C[1 1]@t132@namespace DoubleStream {
      | template < int NSamples, int ShiftAcc, bool DiscardSample, bool SwapRead > class FIR_MultiKernel_cincout;
      | }
      ClassDecl=|
      | namespace DoubleStream {
      | template < int NSamples, int ShiftAcc, bool DiscardSample, bool SwapRead > class FIR_MultiKernel_cincout;
      | }
  filter14 : aieBasic/AIE Class Kernel  KernelAllAttrs=|  PortNames={'sin1'; 'sin2'; 'cin'; 'cout'}  PortSerializedTypes={'{Q2{P{Tinput_stream{1{t{Scint16}}}}}}'; '{Q2{P{Tinput_stream{1{t{Scint16}}}}}}'; '{P{Tinput_stream{1{t{Scacc48_t}}}}}'; '{P{Toutput_stream{1{t{Scacc48_t}}}}}'}  PortWindowSizes={0.000000000000000000e+00; 0.000000000000000000e+00; 0.000000000000000000e+00; 0.000000000000000000e+00}  PortWindowMargins={0.000000000000000000e+00; 0.000000000000000000e+00; 0.000000000000000000e+00; 0.000000000000000000e+00}  PortSynchronicities={'auto', 'auto', 'auto', 'auto'}  PortSignalSizes={0.000000000000000000e+00; 0.000000000000000000e+00; 0.000000000000000000e+00; 8.000000000000000000e+00}  ClassTemplateSpecKind=implicit  ClassTemplateParamNames={'NSamples'; 'ShiftAcc'; 'DiscardSample'; 'SwapRead'}  ClassTemplateParamKinds={'nontype'; 'nontype'; 'nontype'; 'nontype'}  ClassTemplateParamTypes={'int'; 'int'; 'bool'; 'bool'}  ClassTemplateParamValues={'512', '15', '0', '0'}  ClassCtorParamNames={'taps'}  ClassCtorParamSerializedTypes={'{R{Q1{C{Scint16}4}}}'}  ClassCtorParamValues={'[-54-21i 102-525i 8773-2748i 342+439i]'}  ClassIndex=1  ClassCtorIndex=1  ClassTabVisible=on  ClassTemplateParamsVisible=on  ClassCtorDeclVisible=on  ClassCtorParamsVisible=on  FunctionTabVisible=on  FunctionDecl=|  PortAttrs={ 'input', 'sin1', 'input_stream_cint16 * restrict', '', '', '', ''; 'input', 'sin2', 'input_stream_cint16 * restrict', '', '', '', ''; 'input', 'cin', 'input_stream< cacc48_t > *', '', '', '', ''; 'output', 'cout', 'output_stream< cacc48_t > *', '', '', '', 'OUTPUT_SIZE' }  PortAttrsEnables={'off', 'off', 'off', 'off', 'off', 'off', 'off';'off', 'off', 'off', 'off', 'off', 'off', 'off';'off', 'off', 'off', 'off', 'off', 'off', 'off';'off', 'off', 'off', 'off', 'off', 'off', 'on'}  SampleTime=-1  ClassDeclTypeOptions=|  ClassDecl=|  ClassTemplateParams={ 'NSamples', 'int', 'BURST_LENGTH'; 'ShiftAcc', 'int', 'SHIFT_ACC'; 'DiscardSample', 'bool', 'FALSE'; 'SwapRead', 'bool', 'FALSE' }  ClassTemplateParamsEnables={'off', 'off', 'on';'off', 'off', 'on';'off', 'off', 'on';'off', 'off', 'on'}  ClassCtorDeclTypeOptions=C[1 1]@t54@FIR_MultiKernel_cincout(cint16 const ( & taps ) [ 4 ])  ClassCtorDecl=FIR_MultiKernel_cincout(cint16 const ( & taps ) [ 4 ])  ClassCtorParams={ 'taps', 'cint16 const ( &) [ 4 ]', 'phi_0' }  KernelHeaderFile=FirDoubleStream.h  KernelClassName=DoubleStream::FIR_MultiKernel_cincout  KernelFunction=filter  KernelSourceFile=FirDoubleStream.cpp  KernelSearchPaths={'$SRC/aie_kernels'}  PreProcOptions={}  blockJsonConstraints="{\"type\":\"constraint\",\"constraintType\":\"location_kernel\",\"sid\":\"795\",\"lhs\":{\"type\":\"location\",\"templParam\":\"kernel\",\"args\":{\"type\":\"kernel\",\"name\":\"DualStreamSSR/SSR8/filter14\",\"sid\":\"795\"}},\"rhs\":{\"type\":\"tile\",\"args\":[{\"type\":\"evaluable\",\"expr\":\"24\",\"value\":24},{\"type\":\"evaluable\",\"expr\":\"1\",\"value\":1}]},\"equality\":true}"
      KernelAllAttrs=|
      | s[12;12;9;9;19;14;21;23;24;21;12;24;26;26;26;27;28;9;21;23;23;23;24;25;14;19;19;29]@FunctionNameDeclFileNamePortNamesPortTypesPortSerializedTypesPortDirectionsPortWindowSizeEnablesPortWindowMarginEnablesPortSynchronicityEnablesPortSignalSizeEnablesFunctionDeclFunctionTemplateSpecKindFunctionTemplateParamNamesFunctionTemplateParamKindsFunctionTemplateParamTypesFunctionTemplateParamValuesFunctionTemplateParamEnablesClassDeclClassTemplateSpecKindClassTemplateParamNamesClassTemplateParamKindsClassTemplateParamTypesClassTemplateParamValuesClassTemplateParamEnablesClassCtorDeclsClassCtorParamNamesClassCtorParamTypesClassCtorParamSerializedTypes[1 1]@C[28 1]@t6@filtert42@../../../aie/aie_kernels/FirDoubleStream.hC[4 1]@t4@sin1t4@sin2t3@cint4@coutC[4 1]@t30@input_stream_cint16 * restrictt30@input_stream_cint16 * restrictt26@input_stream< cacc48_t > *t27@output_stream< cacc48_t > *C[4 1]@t37@{Q2{P{Tinput_stream{1{t{Scint16}}}}}}t37@{Q2{P{Tinput_stream{1{t{Scint16}}}}}}t35@{P{Tinput_stream{1{t{Scacc48_t}}}}}t36@{P{Toutput_stream{1{t{Scacc48_t}}}}}C[4 1]@t5@inputt5@inputt5@inputt6@outputC[4 1]@l0@l0@l0@l0@C[4 1]@l0@l0@l0@l0@C[4 1]@l0@l0@l0@l0@C[4 1]@l0@l0@l0@l1@t281@namespace DoubleStream {
      | template < int NSamples, int ShiftAcc, bool DiscardSample, bool SwapRead > 
      | void FIR_MultiKernel_cincout::
      | filter(input_stream_cint16 * restrict sin1, input_stream_cint16 * restrict sin2, input_stream< cacc48_t > * cin, output_stream< cacc48_t > * cout);
      | }t4@nonee[0 1]@e[0 1]@e[0 1]@e[0 1]@e[0 1]@t132@namespace DoubleStream {
      | template < int NSamples, int ShiftAcc, bool DiscardSample, bool SwapRead > class FIR_MultiKernel_cincout;
      | }t8@implicitC[4 1]@t8@NSamplest8@ShiftAcct13@DiscardSamplet8@SwapReadC[4 1]@t7@nontypet7@nontypet7@nontypet7@nontypeC[4 1]@t3@intt3@intt4@boolt4@boolC[4 1]@nnnnC[4 1]@l1@l1@l1@l1@C[1 1]@t54@FIR_MultiKernel_cincout(cint16 const ( & taps ) [ 4 ])C[1 1]@C[1 1]@t4@tapsC[1 1]@C[1 1]@t23@cint16 const ( &) [ 4 ]C[1 1]@C[1 1]@t20@{R{Q1{C{Scint16}4}}}
      FunctionDecl=|
      | namespace DoubleStream {
      | template < int NSamples, int ShiftAcc, bool DiscardSample, bool SwapRead > 
      | void FIR_MultiKernel_cincout::
      | filter(input_stream_cint16 * restrict sin1, input_stream_cint16 * restrict sin2, input_stream< cacc48_t > * cin, output_stream< cacc48_t > * cout);
      | }
      ClassDeclTypeOptions=|
      | C[1 1]@t132@namespace DoubleStream {
      | template < int NSamples, int ShiftAcc, bool DiscardSample, bool SwapRead > class FIR_MultiKernel_cincout;
      | }
      ClassDecl=|
      | namespace DoubleStream {
      | template < int NSamples, int ShiftAcc, bool DiscardSample, bool SwapRead > class FIR_MultiKernel_cincout;
      | }
